simulink model "ModeInputHandle"  (R2018b)
settings: Solver=FixedStepDiscrete  StartTime=0.0  StopTime=10.0  FixedStep=0.01  RelTol=1e-3
undefined symbols (not defined in the file or in its folder): c, CmprtMdHMIReqExt2Tp1, CmprtMdHMIReqExtTp1, CmprtMdHMIReqTp1, d, e, EZESwReq1, f, g, IfVeSMSeStNumConfig, j, KeSMSuButtonLongPressedThrshldTm_Val, KeSMSuFoldType_Val, KeSMSwSeatSMSSeatMdTrigGapTimer_Val, KeSMSwSeatTrigWaitTimer_Val, KeSMSwSRSActiveValidTm_Val, LckUlckActvtFunc1, LstLckFunc1, LugSelectSw1, MdReqTp1, PowerMode1, SeatOccupiedSts1, SRSMode1, StPassCmprtMdCtrl_Md10_VCUConfig_Val, StPassCmprtMdCtrl_Md11_VCUConfig_Val, StPassCmprtMdCtrl_Md12_VCUConfig_Val, StPassCmprtMdCtrl_Md13_VCUConfig_Val, StPassCmprtMdCtrl_Md1_VCUConfig_Val, StPassCmprtMdCtrl_Md27_VCUConfig_Val, StPassCmprtMdCtrl_Md28_VCUConfig_Val, StPassCmprtMdCtrl_Md29_VCUConfig_Val, StPassCmprtMdCtrl_Md2_VCUConfig_Val, StPassCmprtMdCtrl_Md30_VCUConfig_Val, StPassCmprtMdCtrl_Md31_VCUConfig_Val, StPassCmprtMdCtrl_Md32_VCUConfig_Val, StPassCmprtMdCtrl_Md3_VCUConfig_Val, StPassCmprtMdCtrl_Md53_VCUConfig_Val, StPassCmprtMdCtrl_Md56_VCUConfig_Val, StPassCmprtMdCtrl_Md57_VCUConfig_Val, StPassCmprtMdCtrl_Md58_VCUConfig_Val, StPassCmprtMdCtrl_Md61_VCUConfig_Val, StPassCmprtMdCtrl_Md62_VCUConfig_Val, StPassCmprtMdCtrl_Md8_VCUConfig_Val, StPassCmprtMdCtrl_Md9_VCUConfig_Val, StSrv_StMd10_Config_Val, StSrv_StMd11_Config_Val, StSrv_StMd12_Config_Val, StSrv_StMd13_Config_Val, StSrv_StMd1_Config_Val, StSrv_StMd27_Config_Val, StSrv_StMd28_Config_Val, StSrv_StMd29_Config_Val, StSrv_StMd2_Config_Val, StSrv_StMd30_Config_Val, StSrv_StMd31_Config_Val, StSrv_StMd32_Config_Val, StSrv_StMd3_Config_Val, StSrv_StMd8_Config_Val, StSrv_StMd9_Config_Val, VehMovState1
libraries: MSMLib x91
(part 1 of 9)
settings Model: PauseTimes=0.13  Creator=su3dcu  LastModifiedBy=su3dcu
settings DataIOCC: SaveFormat=StructureWithTime  ReturnWorkspaceOutputs=on
settings OptimizationCC: DefaultParameterBehavior=Inlined  EnhancedBackFolding=on  PassReuseOutputArgsAs=Individual arguments  ZeroExternalMemoryAtStartup=off  ZeroInternalMemoryAtStartup=off  OptimizeBlockOrder=speed  DifferentSizesBufferReuse=on  OptimizationCustomize=off
settings DebuggingCC: ParameterTunabilityLossMsg=error
settings HardwareCC: ProdLongLongMode=on
settings ModelReferenceCC: ModelReferenceNumInstancesAllowed=Single
settings SFSimCC: SimCustomHeaderCode="#include\"Rte_Type.h\""  MATLABDynamicMemAlloc=off
settings RTWCC: SystemTargetFile=autosar.tlc  GenCodeOnly=on  TemplateMakefile=ert_default_tmf  Description=AUTOSAR  GenerateReport=on  BuildConfiguration=Debug  IncludeHyperlinkInReport=on  LaunchReport=on  CodeExecutionProfiling=on  GenerateTraceInfo=on  GenerateTraceReport=on  GenerateTraceReportSl=on  GenerateTraceReportSf=on  GenerateTraceReportEml=on  GenerateCodeMetricsReport=on
settings CodeAppCC: ForceParamTrailComments=on  IgnoreCustomStorageClasses=off  MaxIdLength=63  OperatorAnnotations=on  SimulinkDataObjDesc=on  SFDataObjDesc=on  InsertBlockDesc=on
settings STFCustomTargetCC: TargetLangStandard=C99 (ISO)  MultiwordLength=256  ParMdlRefBuildCompliant=on  CompOptLevelCompliant=on  IncludeMdlTerminateFcn=off  CombineOutputUpdateFcns=on  SuppressErrorStatus=on  ERTCustomFileBanners=on  SupportAbsoluteTime=off  PurelyIntegerCode=on  SupportNonFinite=off  SupportComplex=off  SupportContinuousTime=off  SupportNonInlinedSFcns=off  RemoveResetFunc=on  MATLABClassNameForMDSCustomization=Simulink.SoftwareTarget.ERTCustomization  AutosarCompliant=on  UseToolchainInfoCompliant=on  LookupTableObjectStructAxisOrder=2,1,3,4,...  LUTObjectStructOrderEvenSpacing=Size,Table,Breakpoints  SystemTargetFile=autosar.tlc
settings ERTTargetCC: TargetLangStandard=C99 (ISO)  ConcurrentExecutionCompliant=off  IncludeMdlTerminateFcn=off  SuppressErrorStatus=on  SupportAbsoluteTime=off  PurelyIntegerCode=on  SupportNonFinite=off  SupportComplex=off  ModelStepFunctionPrototypeControlCompliant=off  CPPClassGenCompliant=off  AutosarCompliant=on  LookupTableObjectStructAxisOrder=2,1,3,4,...  LUTObjectStructOrderEvenSpacing=Size,Table,Breakpoints  InlinedParameterPlacement=NonHierarchical  ERTCustomFileTemplate=example_file_process.tlc  ERTFilePackagingFormat=Compact
settings ConfigComp: DVTestSuiteOptimization=CombinedObjectives (Nonlinear Extended)  DVDetectActiveLogic=on  DVDetectOutOfBounds=on

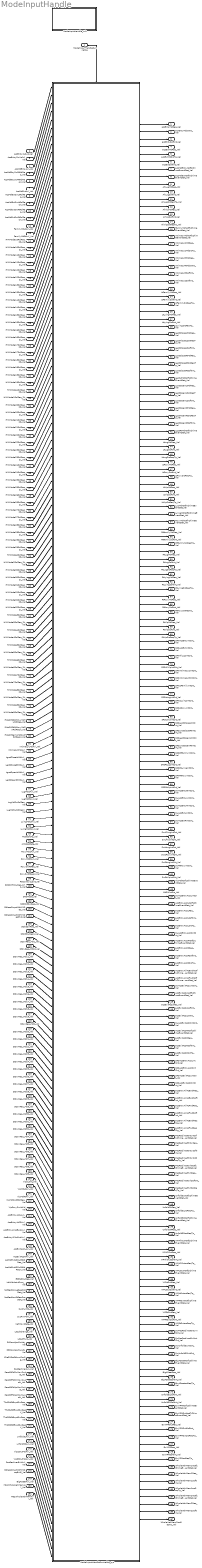
== system ModeInputHandle ==
  ModelInputHandleRunnable : Inport  SampleTime=0.01  OutputFunctionCall=on
  AcsEntry2LSwt_Val : Inport  Port=2  OutDataTypeStr=uint8  PortDimensions=1
  AcsEntrySwValid_Val : Inport  Port=3  OutDataTypeStr=uint8  PortDimensions=1
  AcsMdEntyAvl_Val : Inport  Port=4  OutDataTypeStr=boolean  PortDimensions=1
  AcsMdEtrySwRtRclReq_Val : Inport  Port=5  OutDataTypeStr=boolean  PortDimensions=1
  AcsMdEtrySwRtRclReqV_Val : Inport  Port=6  OutDataTypeStr=boolean  PortDimensions=1
  AcsMdExtAvl_Val : Inport  Port=7  OutDataTypeStr=boolean  PortDimensions=1
  AcsMdExtSwLtRclReq_Val : Inport  Port=8  OutDataTypeStr=boolean  PortDimensions=1
  AcsMdExtSwLtRclReqV_Val : Inport  Port=9  OutDataTypeStr=uint8  PortDimensions=1
  AcsMdExtSwRtRclReq_Val : Inport  Port=10  OutDataTypeStr=boolean  PortDimensions=1
  AcsMdExtSwRtRclReqV_Val : Inport  Port=11  OutDataTypeStr=boolean  PortDimensions=1
  FamilyMdLtAvl_Val : Inport  Port=12  OutDataTypeStr=boolean  PortDimensions=1
  FamilyMdRtAvl_Val : Inport  Port=13  OutDataTypeStr=boolean  PortDimensions=1
  HMIMode10RclReq_2R_Val : Inport  Port=14  OutDataTypeStr=Enum: MdReqTp1  PortDimensions=1
  HMIMode10RclReq_2L_Val : Inport  Port=15  OutDataTypeStr=Enum: MdReqTp1  PortDimensions=1
  HMIMode11RclReq_2R_Val : Inport  Port=16  OutDataTypeStr=Enum: MdReqTp1  PortDimensions=1
  HMIMode11RclReq_2L_Val : Inport  Port=17  OutDataTypeStr=Enum: MdReqTp1  PortDimensions=1
  HMIMode12RclReq_2R_Val : Inport  Port=18  OutDataTypeStr=Enum: MdReqTp1  PortDimensions=1
  HMIMode12RclReq_2L_Val : Inport  Port=19  OutDataTypeStr=Enum: MdReqTp1  PortDimensions=1
  HMIMode13RclReq_2R_Val : Inport  Port=20  OutDataTypeStr=Enum: MdReqTp1  PortDimensions=1
  HMIMode13RclReq_2L_Val : Inport  Port=21  OutDataTypeStr=Enum: MdReqTp1  PortDimensions=1
  HMIMode14RclReq_2R_Val : Inport  Port=22  OutDataTypeStr=Enum: MdReqTp1  PortDimensions=1
  HMIMode14RclReq_2L_Val : Inport  Port=23  OutDataTypeStr=Enum: MdReqTp1  PortDimensions=1
  HMIMode15RclReq_2R_Val : Inport  Port=24  OutDataTypeStr=Enum: MdReqTp1  PortDimensions=1
  HMIMode15RclReq_2L_Val : Inport  Port=25  OutDataTypeStr=Enum: MdReqTp1  PortDimensions=1
  HMIMode16RclReq_2R_Val : Inport  Port=26  OutDataTypeStr=Enum: MdReqTp1  PortDimensions=1
  HMIMode16RclReq_2L_Val : Inport  Port=27  OutDataTypeStr=Enum: MdReqTp1  PortDimensions=1
  HMIMode17RclReq_2R_Val : Inport  Port=28  OutDataTypeStr=Enum: MdReqTp1  PortDimensions=1
  HMIMode17RclReq_2L_Val : Inport  Port=29  OutDataTypeStr=Enum: MdReqTp1  PortDimensions=1
  HMIMode18RclReq_2R_Val : Inport  Port=30  OutDataTypeStr=Enum: MdReqTp1  PortDimensions=1
  HMIMode18RclReq_2L_Val : Inport  Port=31  OutDataTypeStr=Enum: MdReqTp1  PortDimensions=1
  HMIMode19RclReq_2R_Val : Inport  Port=32  OutDataTypeStr=Enum: MdReqTp1  PortDimensions=1
  HMIMode19RclReq_2L_Val : Inport  Port=33  OutDataTypeStr=Enum: MdReqTp1  PortDimensions=1
  HMIMode1RclReq_2R_Val : Inport  Port=34  OutDataTypeStr=Enum: MdReqTp1  PortDimensions=1
  HMIMode1RclReq_2L_Val : Inport  Port=35  OutDataTypeStr=Enum: MdReqTp1  PortDimensions=1
  HMIMode20RclReq_2R_Val : Inport  Port=36  OutDataTypeStr=Enum: MdReqTp1  PortDimensions=1
  HMIMode20RclReq_2L_Val : Inport  Port=37  OutDataTypeStr=Enum: MdReqTp1  PortDimensions=1
  HMIMode21RclReq_2R_Val : Inport  Port=38  OutDataTypeStr=Enum: MdReqTp1  PortDimensions=1
  HMIMode21RclReq_2L_Val : Inport  Port=39  OutDataTypeStr=Enum: MdReqTp1  PortDimensions=1
  HMIMode22RclReq_2R_Val : Inport  Port=40  OutDataTypeStr=Enum: MdReqTp1  PortDimensions=1
  HMIMode22RclReq_2L_Val : Inport  Port=41  OutDataTypeStr=Enum: MdReqTp1  PortDimensions=1
  HMIMode23RclReq_2R_Val : Inport  Port=42  OutDataTypeStr=Enum: MdReqTp1  PortDimensions=1
  HMIMode23RclReq_2L_Val : Inport  Port=43  OutDataTypeStr=Enum: MdReqTp1  PortDimensions=1
  HMIMode24RclReq_2R_Val : Inport  Port=44  OutDataTypeStr=Enum: MdReqTp1  PortDimensions=1
  HMIMode24RclReq_2L_Val : Inport  Port=45  OutDataTypeStr=Enum: MdReqTp1  PortDimensions=1
  HMIMode25RclReq_2R_Val : Inport  Port=46  OutDataTypeStr=Enum: MdReqTp1  PortDimensions=1
  HMIMode25RclReq_2L_Val : Inport  Port=47  OutDataTypeStr=Enum: MdReqTp1  PortDimensions=1
  HMIMode26RclReq_2R_Val : Inport  Port=48  OutDataTypeStr=Enum: MdReqTp1  PortDimensions=1
  HMIMode26RclReq_2L_Val : Inport  Port=49  OutDataTypeStr=Enum: MdReqTp1  PortDimensions=1
  HMIMode27RclReq_2R_Val : Inport  Port=50  OutDataTypeStr=Enum: MdReqTp1  PortDimensions=1
  HMIMode27RclReq_2L_Val : Inport  Port=51  OutDataTypeStr=Enum: MdReqTp1  PortDimensions=1
  HMIMode28RclReq_2R_Val : Inport  Port=52  OutDataTypeStr=Enum: MdReqTp1  PortDimensions=1
  HMIMode28RclReq_2L_Val : Inport  Port=53  OutDataTypeStr=Enum: MdReqTp1  PortDimensions=1
  HMIMode29RclReq_2R_Val : Inport  Port=54  OutDataTypeStr=Enum: MdReqTp1  PortDimensions=1
  HMIMode29RclReq_2L_Val : Inport  Port=55  OutDataTypeStr=Enum: MdReqTp1  PortDimensions=1
  HMIMode2RclReq_2R_Val : Inport  Port=56  OutDataTypeStr=Enum: MdReqTp1  PortDimensions=1
  HMIMode2RclReq_2L_Val : Inport  Port=57  OutDataTypeStr=Enum: MdReqTp1  PortDimensions=1
  HMIMode30RclReq_2R_Val : Inport  Port=58  OutDataTypeStr=Enum: MdReqTp1  PortDimensions=1
  HMIMode30RclReq_2L_Val : Inport  Port=59  OutDataTypeStr=Enum: MdReqTp1  PortDimensions=1
  HMIMode31RclReq_2R_Val : Inport  Port=60  OutDataTypeStr=Enum: MdReqTp1  PortDimensions=1
  HMIMode31RclReq_2L_Val : Inport  Port=61  OutDataTypeStr=Enum: MdReqTp1  PortDimensions=1
  HMIMode32RclReq_2R_Val : Inport  Port=62  OutDataTypeStr=Enum: MdReqTp1  PortDimensions=1
  HMIMode32RclReq_2L_Val : Inport  Port=63  OutDataTypeStr=Enum: MdReqTp1  PortDimensions=1
  HMIMode3RclReq_2R_Val : Inport  Port=64  OutDataTypeStr=Enum: MdReqTp1  PortDimensions=1
  HMIMode3RclReq_2L_Val : Inport  Port=65  OutDataTypeStr=Enum: MdReqTp1  PortDimensions=1
  HMIMode4RclReq_2R_Val : Inport  Port=66  OutDataTypeStr=Enum: MdReqTp1  PortDimensions=1
  HMIMode4RclReq_2L_Val : Inport  Port=67  OutDataTypeStr=Enum: MdReqTp1  PortDimensions=1
  HMIMode5RclReq_2R_Val : Inport  Port=68  OutDataTypeStr=Enum: MdReqTp1  PortDimensions=1
  HMIMode5RclReq_2L_Val : Inport  Port=69  OutDataTypeStr=Enum: MdReqTp1  PortDimensions=1
  HMIMode6RclReq_2R_Val : Inport  Port=70  OutDataTypeStr=Enum: MdReqTp1  PortDimensions=1
  HMIMode6RclReq_2L_Val : Inport  Port=71  OutDataTypeStr=Enum: MdReqTp1  PortDimensions=1
  HMIMode7RclReq_2R_Val : Inport  Port=72  OutDataTypeStr=Enum: MdReqTp1  PortDimensions=1
  HMIMode7RclReq_2L_Val : Inport  Port=73  OutDataTypeStr=Enum: MdReqTp1  PortDimensions=1
  HMIMode8RclReq_2R_Val : Inport  Port=74  OutDataTypeStr=Enum: MdReqTp1  PortDimensions=1
  HMIMode8RclReq_2L_Val : Inport  Port=75  OutDataTypeStr=Enum: MdReqTp1  PortDimensions=1
  HMIMode9RclReq_2R_Val : Inport  Port=76  OutDataTypeStr=Enum: MdReqTp1  PortDimensions=1
  HMIMode9RclReq_2L_Val : Inport  Port=77  OutDataTypeStr=Enum: MdReqTp1  PortDimensions=1
  IfVeSMSbRrRcvyMdSwRclReq_Val : Inport  Port=78  OutDataTypeStr=uint8  PortDimensions=1
  IfVeSMSbRrRcvyMdSwRclReqV_Val : Inport  Port=79  OutDataTypeStr=boolean  PortDimensions=1
  IfVeSMSeVipMdSwRtRclReqV_Val : Inport  Port=80  OutDataTypeStr=boolean  PortDimensions=1
  IntimacyLMdAvl_Val : Inport  Port=81  OutDataTypeStr=boolean  PortDimensions=1
  IntimacyRMdAvl_Val : Inport  Port=82  OutDataTypeStr=boolean  PortDimensions=1
  LgrstCloseLtMdAvl_Val : Inport  Port=83  OutDataTypeStr=boolean  PortDimensions=1
  LgrstCloseRtMdAvl_Val : Inport  Port=84  OutDataTypeStr=boolean  PortDimensions=1
  LgrstOpenLtMdAvl_Val : Inport  Port=85  OutDataTypeStr=boolean  PortDimensions=1
  LgrstOpenRtMdAvl_Val : Inport  Port=86  OutDataTypeStr=boolean  PortDimensions=1
  LugMdLtAvl_Val : Inport  Port=87  OutDataTypeStr=boolean  PortDimensions=1
  LugMdRtAvl_Val : Inport  Port=88  OutDataTypeStr=boolean  PortDimensions=1
  LugMdSwRclReq_Val : Inport  Port=89  OutDataTypeStr=boolean  PortDimensions=1
  LugMdSwRclReqV_Val : Inport  Port=90  OutDataTypeStr=uint8  PortDimensions=1
  LyingMdLtAvl_Val : Inport  Port=91  OutDataTypeStr=boolean  PortDimensions=1
  LyingMdRtAvl_Val : Inport  Port=92  OutDataTypeStr=boolean  PortDimensions=1
  ModeSrcTp_Val : Inport  Port=93  OutDataTypeStr=Enum: SrcReqTp1  PortDimensions=1
  oModeState_Val : Inport  Port=94  OutDataTypeStr=Enum: MdTp1  PortDimensions=1
  RcvyMdLtAvl_Val : Inport  Port=95  OutDataTypeStr=boolean  PortDimensions=1
  RcvyMdRtAvl_Val : Inport  Port=96  OutDataTypeStr=boolean  PortDimensions=1
  RcvySwRtReq_Val : Inport  Port=97  OutDataTypeStr=boolean  PortDimensions=1
  RcvySwRtReqV_Val : Inport  Port=98  OutDataTypeStr=boolean  PortDimensions=1
  Recovery2LSwt_Val : Inport  Port=99  OutDataTypeStr=uint8  PortDimensions=1
  SRSCnfmSwReq_67_2_Val : Inport  Port=100  OutDataTypeStr=boolean  PortDimensions=1
  SRSMode_Val : Inport  Port=101  OutDataTypeStr=Enum: SRSCurMode1  PortDimensions=1
  SRSSlctSwReq_Val : Inport  Port=102  OutDataTypeStr=Enum: SRSMode1  PortDimensions=1
  StPassCmprtMdHMIReq_Val : Inport  Port=103  OutDataTypeStr=Enum: CmprtMdHMIReqTp1  PortDimensions=1
  StPassCmprtMdHMIReqExt_Val : Inport  Port=104  OutDataTypeStr=Enum: CmprtMdHMIReqExtTp1  PortDimensions=1
  StSlctSwReq_Val : Inport  Port=105  OutDataTypeStr=Enum: LugSelectSw1  PortDimensions=1
  StSlctSwReqV_Val : Inport  Port=106  OutDataTypeStr=boolean  PortDimensions=1
  StSrvReq_Md1_Val : Inport  Port=107  OutDataTypeStr=boolean  PortDimensions=1
  StSrvReq_Md10_Val : Inport  Port=108  OutDataTypeStr=boolean  PortDimensions=1
  StSrvReq_Md11_Val : Inport  Port=109  OutDataTypeStr=boolean  PortDimensions=1
  StSrvReq_Md12_Val : Inport  Port=110  OutDataTypeStr=boolean  PortDimensions=1
  StSrvReq_Md13_Val : Inport  Port=111  OutDataTypeStr=boolean  PortDimensions=1
  StSrvReq_Md14_Val : Inport  Port=112  OutDataTypeStr=boolean  PortDimensions=1
  StSrvReq_Md15_Val : Inport  Port=113  OutDataTypeStr=boolean  PortDimensions=1
  StSrvReq_Md16_Val : Inport  Port=114  OutDataTypeStr=boolean  PortDimensions=1
  StSrvReq_Md17_Val : Inport  Port=115  OutDataTypeStr=boolean  PortDimensions=1
  StSrvReq_Md18_Val : Inport  Port=116  OutDataTypeStr=boolean  PortDimensions=1
  StSrvReq_Md19_Val : Inport  Port=117  OutDataTypeStr=boolean  PortDimensions=1
  StSrvReq_Md2_Val : Inport  Port=118  OutDataTypeStr=boolean  PortDimensions=1
  StSrvReq_Md20_Val : Inport  Port=119  OutDataTypeStr=boolean  PortDimensions=1
  StSrvReq_Md21_Val : Inport  Port=120  OutDataTypeStr=boolean  PortDimensions=1
  StSrvReq_Md22_Val : Inport  Port=121  OutDataTypeStr=boolean  PortDimensions=1
  StSrvReq_Md23_Val : Inport  Port=122  OutDataTypeStr=boolean  PortDimensions=1
  StSrvReq_Md24_Val : Inport  Port=123  OutDataTypeStr=boolean  PortDimensions=1
  StSrvReq_Md25_Val : Inport  Port=124  OutDataTypeStr=boolean  PortDimensions=1
  StSrvReq_Md26_Val : Inport  Port=125  OutDataTypeStr=boolean  PortDimensions=1
  StSrvReq_Md27_Val : Inport  Port=126  OutDataTypeStr=boolean  PortDimensions=1
  StSrvReq_Md28_Val : Inport  Port=127  OutDataTypeStr=boolean  PortDimensions=1
  StSrvReq_Md29_Val : Inport  Port=128  OutDataTypeStr=boolean  PortDimensions=1
  StSrvReq_Md3_Val : Inport  Port=129  OutDataTypeStr=boolean  PortDimensions=1
  StSrvReq_Md30_Val : Inport  Port=130  OutDataTypeStr=boolean  PortDimensions=1
  StSrvReq_Md31_Val : Inport  Port=131  OutDataTypeStr=boolean  PortDimensions=1
  StSrvReq_Md32_Val : Inport  Port=132  OutDataTypeStr=boolean  PortDimensions=1
  StSrvReq_Md4_Val : Inport  Port=133  OutDataTypeStr=boolean  PortDimensions=1
  StSrvReq_Md5_Val : Inport  Port=134  OutDataTypeStr=boolean  PortDimensions=1
  StSrvReq_Md6_Val : Inport  Port=135  OutDataTypeStr=boolean  PortDimensions=1
  StSrvReq_Md7_Val : Inport  Port=136  OutDataTypeStr=boolean  PortDimensions=1
  StSrvReq_Md8_Val : Inport  Port=137  OutDataTypeStr=boolean  PortDimensions=1
  StSrvReq_Md9_Val : Inport  Port=138  OutDataTypeStr=boolean  PortDimensions=1
  Vip2LSwt_Val : Inport  Port=139  OutDataTypeStr=uint8  PortDimensions=1
  VipMdLtAvl_Val : Inport  Port=140  OutDataTypeStr=boolean  PortDimensions=1
  VipMdRtAvl_Val : Inport  Port=141  OutDataTypeStr=boolean  PortDimensions=1
  VipMdSwRtRclReq_Val : Inport  Port=142  OutDataTypeStr=boolean  PortDimensions=1
  VipRcvySwValid_Val : Inport  Port=143  OutDataTypeStr=uint8  PortDimensions=1
  AcsEntry4s2LAvl_Val : Inport  Port=144  OutDataTypeStr=boolean  PortDimensions=1
  AcsEntry4s2RAvl_Val : Inport  Port=145  OutDataTypeStr=boolean  PortDimensions=1
  AcsEntryAll4sBwdAvl_Val : Inport  Port=146  OutDataTypeStr=boolean  PortDimensions=1
  AcsEntryAll4sFwdAvl_Val : Inport  Port=147  OutDataTypeStr=boolean  PortDimensions=1
  AcsExit4s2LAvl_Val : Inport  Port=148  OutDataTypeStr=boolean  PortDimensions=1
  AcsExit4s2RAvl_Val : Inport  Port=149  OutDataTypeStr=boolean  PortDimensions=1
  AcsMdExt4SSwRtRclReq_Val : Inport  Port=150  OutDataTypeStr=boolean  PortDimensions=1
  AcsMdExt4SSwRtRclReqV_Val : Inport  Port=151  OutDataTypeStr=boolean  PortDimensions=1
  EZE4SSwReq_Val : Inport  Port=152  OutDataTypeStr=Enum: EZESwReq1  PortDimensions=1
  LckUlckActvtFunc_Val : Inport  Port=153  OutDataTypeStr=Enum: LckUlckActvtFunc1  PortDimensions=1
  NotSecRowLeSeaOccStat_Val : Inport  Port=154  OutDataTypeStr=Enum: SeatOccupiedSts1  PortDimensions=1
  NotSecRowRtSeaOccStat_Val : Inport  Port=155  OutDataTypeStr=Enum: SeatOccupiedSts1  PortDimensions=1
  SysPwrMd_Val : Inport  Port=156  OutDataTypeStr=Enum: PowerMode1  PortDimensions=1
  SysPwrMdV_Val : Inport  Port=157  OutDataTypeStr=boolean  PortDimensions=1
  VehMovState_Val : Inport  Port=158  OutDataTypeStr=Enum: VehMovState1  PortDimensions=1
  LstLckChange_Val : Inport  Port=159  OutDataTypeStr=uint8  PortDimensions=1
  LstLckFunc_Val : Inport  Port=160  OutDataTypeStr=Enum: LstLckFunc1  PortDimensions=1
  RLDoorAjarSwAct_Val : Inport  Port=161  OutDataTypeStr=boolean  PortDimensions=1
  RRDoorAjarSwAct_Val : Inport  Port=162  OutDataTypeStr=boolean  PortDimensions=1
  IfVeSMSeStNumConfig_Val : Inport  Port=163  OutDataTypeStr=Enum: IfVeSMSeStNumConfig  PortDimensions=1
  PasReclinerAvl_Val : Inport  Port=164  OutDataTypeStr=boolean  PortDimensions=1
  PassStFldDnMovSwAct_Val : Inport  Port=165  OutDataTypeStr=boolean  PortDimensions=1
  PassStFldDnMovSwActV_Val : Inport  Port=166  OutDataTypeStr=boolean  PortDimensions=1
  PassStFldUpMovSwAct_Val : Inport  Port=167  OutDataTypeStr=boolean  PortDimensions=1
  PassStFldUpMovSwActV_Val : Inport  Port=168  OutDataTypeStr=boolean  PortDimensions=1
  ThdRLtStExpdSwReq_Val : Inport  Port=169  OutDataTypeStr=boolean  PortDimensions=1
  ThdRLtStExpdSwReqV_Val : Inport  Port=170  OutDataTypeStr=boolean  PortDimensions=1
  ThdRRtStExpdSwReq_Val : Inport  Port=171  OutDataTypeStr=boolean  PortDimensions=1
  ThdRRtStExpdSwReqV_Val : Inport  Port=172  OutDataTypeStr=boolean  PortDimensions=1
  unfold3LAvl_Val : Inport  Port=173  OutDataTypeStr=boolean  PortDimensions=1
  unfold3RAvl_Val : Inport  Port=174  OutDataTypeStr=boolean  PortDimensions=1
  VipLtOutMdAvl_Val : Inport  Port=175  OutDataTypeStr=boolean  PortDimensions=1
  VipRtOutMdAvl_Val : Inport  Port=176  OutDataTypeStr=boolean  PortDimensions=1
  PasReclinerExitAvl_Val : Inport  Port=177  OutDataTypeStr=boolean  PortDimensions=1
  StPassCmprtMdHMIReqExt2_Val : Inport  Port=178  OutDataTypeStr=Enum: CmprtMdHMIReqExt2Tp1  PortDimensions=1
  Big4SeatAvl_Val : Inport  Port=179  OutDataTypeStr=boolean  PortDimensions=1
  M61WholeVehMemAvl_Val : Inport  Port=180  OutDataTypeStr=boolean  PortDimensions=1
  M62WholeVehMemAvl_Val : Inport  Port=181  OutDataTypeStr=boolean  PortDimensions=1
  ModeInputHandle_Init : Subsystem
  ModelInputHandleRunnable_sys : Subsystem
  acsEntyMdReq_Val : Outport  OutDataTypeStr=boolean  PortDimensions=1
  acsEntyMdSrcTp_Val : Outport  Port=2  OutDataTypeStr=Enum: SrcReqTp1  PortDimensions=1
  acsEntySoftInt_Val : Outport  Port=3  OutDataTypeStr=IntEnable  PortDimensions=1
  acsExtMdReq_Val : Outport  Port=4  OutDataTypeStr=boolean  PortDimensions=1
  acsExtMdSrcTp_Val : Outport  Port=5  OutDataTypeStr=Enum: SrcReqTp1  PortDimensions=1
  acsExtSoftInt_Val : Outport  Port=6  OutDataTypeStr=IntEnable  PortDimensions=1
  acsMdEntryNotf1ChimeEventStat_Val : Outport  Port=7  OutDataTypeStr=boolean  PortDimensions=1
  acsMdExtNotf1ChimeEventStat_Val : Outport  Port=8  OutDataTypeStr=boolean  PortDimensions=1
  AllLugMdReq_Val : Outport  Port=9  OutDataTypeStr=boolean  PortDimensions=1
  AllLugSoftInt_Val : Outport  Port=10  OutDataTypeStr=IntEnable  PortDimensions=1
  AllLugSrcReqTp_Val : Outport  Port=11  OutDataTypeStr=Enum: SrcReqTp1  PortDimensions=1
  AllVipMdReq_Val : Outport  Port=12  OutDataTypeStr=boolean  PortDimensions=1
  AllVipSoftInt_Val : Outport  Port=13  OutDataTypeStr=IntEnable  PortDimensions=1
  AllVipSrcReqTp_Val : Outport  Port=14  OutDataTypeStr=Enum: SrcReqTp1  PortDimensions=1
  FamilyMdNotf1ChimeEventStat_Val : Outport  Port=15  OutDataTypeStr=boolean  PortDimensions=1
  IntimacyMdNotf1ChimeEventStat_Val : Outport  Port=16  OutDataTypeStr=boolean  PortDimensions=1
  IntimacyLtMdReq_Val : Outport  Port=17  OutDataTypeStr=boolean  PortDimensions=1
  IntimacyLtMdSrcTp_Val : Outport  Port=18  OutDataTypeStr=Enum: SrcReqTp1  PortDimensions=1
  IntimacyRtMdReq_Val : Outport  Port=19  OutDataTypeStr=boolean  PortDimensions=1
  IntimacyRtMdSrcTp_Val : Outport  Port=20  OutDataTypeStr=Enum: SrcReqTp1  PortDimensions=1
  IntimacyRtSoftInt_Val : Outport  Port=21  OutDataTypeStr=IntEnable  PortDimensions=1
  IntimacyLtSoftInt_Val : Outport  Port=22  OutDataTypeStr=IntEnable  PortDimensions=1
  LtFamilyMdReq_Val : Outport  Port=23  OutDataTypeStr=boolean  PortDimensions=1
  LtFamilySoftInt_Val : Outport  Port=24  OutDataTypeStr=IntEnable  PortDimensions=1
  LtFamilySrcReqTp_Val : Outport  Port=25  OutDataTypeStr=Enum: SrcReqTp1  PortDimensions=1
  LtLyingMdReq_Val : Outport  Port=26  OutDataTypeStr=boolean  PortDimensions=1
  LtLyingSoftInt_Val : Outport  Port=27  OutDataTypeStr=IntEnable  PortDimensions=1
  LtLyingSrcReqTp_Val : Outport  Port=28  OutDataTypeStr=Enum: SrcReqTp1  PortDimensions=1
  LgrstCloseLtMdReq_Val : Outport  Port=29  OutDataTypeStr=boolean  PortDimensions=1
  LgrstCloseLtSrcReqTp_Val : Outport  Port=30  OutDataTypeStr=Enum: SrcReqTp1  PortDimensions=1
  LgrstCloseLtSoftInt_Val : Outport  Port=31  OutDataTypeStr=IntEnable  PortDimensions=1
  LgrstCloseRtMdReq_Val : Outport  Port=32  OutDataTypeStr=boolean  PortDimensions=1
  LgrstCloseRtSrcReqTp_Val : Outport  Port=33  OutDataTypeStr=Enum: SrcReqTp1  PortDimensions=1
  LgrstCloseRtSoftInt_Val : Outport  Port=34  OutDataTypeStr=IntEnable  PortDimensions=1
  LgrstLtMdNotf1ChimeEventStat_Val : Outport  Port=35  OutDataTypeStr=boolean  PortDimensions=1
  LgrstOpenLtMdReq_Val : Outport  Port=36  OutDataTypeStr=boolean  PortDimensions=1
  LgrstOpenLtSrcReqTp_Val : Outport  Port=37  OutDataTypeStr=Enum: SrcReqTp1  PortDimensions=1
  LgrstOpenLtSoftInt_Val : Outport  Port=38  OutDataTypeStr=IntEnable  PortDimensions=1
  LgrstOpenRtMdReq_Val : Outport  Port=39  OutDataTypeStr=boolean  PortDimensions=1
  LgrstOpenRtSrcReqTp_Val : Outport  Port=40  OutDataTypeStr=Enum: SrcReqTp1  PortDimensions=1
  LgrstOpenRtSoftInt_Val : Outport  Port=41  OutDataTypeStr=IntEnable  PortDimensions=1
  LgrstRtMdNotf1ChimeEventStat_Val : Outport  Port=42  OutDataTypeStr=boolean  PortDimensions=1
  LtLugMdReq_Val : Outport  Port=43  OutDataTypeStr=boolean  PortDimensions=1
  LtLugSoftInt_Val : Outport  Port=44  OutDataTypeStr=IntEnable  PortDimensions=1
  LtLugSrcReqTp_Val : Outport  Port=45  OutDataTypeStr=Enum: SrcReqTp1  PortDimensions=1
  LtRcvyMdReq_Val : Outport  Port=46  OutDataTypeStr=boolean  PortDimensions=1
  LtRcvySoftInt_Val : Outport  Port=47  OutDataTypeStr=IntEnable  PortDimensions=1
  LtRcvySrcReqTp_Val : Outport  Port=48  OutDataTypeStr=Enum: SrcReqTp1  PortDimensions=1
  LtVipMdReq_Val : Outport  Port=49  OutDataTypeStr=boolean  PortDimensions=1
  LtVipSoftInt_Val : Outport  Port=50  OutDataTypeStr=IntEnable  PortDimensions=1
  LtVipSrcReqTp_Val : Outport  Port=51  OutDataTypeStr=Enum: SrcReqTp1  PortDimensions=1
  LugMdNotf1ChimeEventStat_Val : Outport  Port=52  OutDataTypeStr=boolean  PortDimensions=1
  LyingMdNotf1ChimeEventStat_Val : Outport  Port=53  OutDataTypeStr=boolean  PortDimensions=1
  RcvyMdNotf1ChimeEventStat_Val : Outport  Port=54  OutDataTypeStr=boolean  PortDimensions=1
  RtFamilyMdReq_Val : Outport  Port=55  OutDataTypeStr=boolean  PortDimensions=1
  RtFamilySoftInt_Val : Outport  Port=56  OutDataTypeStr=IntEnable  PortDimensions=1
  RtFamilySrcReqTp_Val : Outport  Port=57  OutDataTypeStr=Enum: SrcReqTp1  PortDimensions=1
  RtLugMdReq_Val : Outport  Port=58  OutDataTypeStr=boolean  PortDimensions=1
  RtLugSoftInt_Val : Outport  Port=59  OutDataTypeStr=IntEnable  PortDimensions=1
  RtLugSrcReqTp_Val : Outport  Port=60  OutDataTypeStr=Enum: SrcReqTp1  PortDimensions=1
  RtLyingMdReq_Val : Outport  Port=61  OutDataTypeStr=boolean  PortDimensions=1
  RtLyingSoftInt_Val : Outport  Port=62  OutDataTypeStr=IntEnable  PortDimensions=1
  RtLyingSrcReqTp_Val : Outport  Port=63  OutDataTypeStr=Enum: SrcReqTp1  PortDimensions=1
  RtRcvyMdReq_Val : Outport  Port=64  OutDataTypeStr=boolean  PortDimensions=1
  RtRcvySoftInt_Val : Outport  Port=65  OutDataTypeStr=IntEnable  PortDimensions=1
  RtRcvySrcReqTp_Val : Outport  Port=66  OutDataTypeStr=Enum: SrcReqTp1  PortDimensions=1
  RtVipMdReq_Val : Outport  Port=67  OutDataTypeStr=boolean  PortDimensions=1
  RtVipSoftInt_Val : Outport  Port=68  OutDataTypeStr=IntEnable  PortDimensions=1
  RtVipSrcReqTp_Val : Outport  Port=69  OutDataTypeStr=Enum: SrcReqTp1  PortDimensions=1
  SRSAcsEntyIntCnt_Val : Outport  Port=70  OutDataTypeStr=IntCnt  PortDimensions=1
  SRSAcsExtIntCnt_Val : Outport  Port=71  OutDataTypeStr=IntCnt  PortDimensions=1
  SRSAllLugIntCnt_Val : Outport  Port=72  OutDataTypeStr=IntCnt  PortDimensions=1
  SRSAllVipIntCnt_Val : Outport  Port=73  OutDataTypeStr=IntCnt  PortDimensions=1
  SRSIntimacyLtIntCnt_Val : Outport  Port=74  OutDataTypeStr=IntCnt  PortDimensions=1
  SRSIntimacyRtIntCnt_Val : Outport  Port=75  OutDataTypeStr=IntCnt  PortDimensions=1
  SRSLtFamilyIntCnt_Val : Outport  Port=76  OutDataTypeStr=IntCnt  PortDimensions=1
  SRSLtLugIntCnt_Val : Outport  Port=77  OutDataTypeStr=IntCnt  PortDimensions=1
  SRSLtLyingIntCnt_Val : Outport  Port=78  OutDataTypeStr=IntCnt  PortDimensions=1
  SRSLtRcvyIntCnt_Val : Outport  Port=79  OutDataTypeStr=IntCnt  PortDimensions=1
  SRSLtVipIntCnt_Val : Outport  Port=80  OutDataTypeStr=IntCnt  PortDimensions=1
  SRSLgrstCloseLtIntCnt_Val : Outport  Port=81  OutDataTypeStr=IntCnt  PortDimensions=1
  SRSLgrstCloseRtIntCnt_Val : Outport  Port=82  OutDataTypeStr=IntCnt  PortDimensions=1
  SRSLgrstOpenLtIntCnt_Val : Outport  Port=83  OutDataTypeStr=IntCnt  PortDimensions=1
  SRSLgrstOpenRtIntCnt_Val : Outport  Port=84  OutDataTypeStr=IntCnt  PortDimensions=1
  SRSRtFamilyIntCnt_Val : Outport  Port=85  OutDataTypeStr=IntCnt  PortDimensions=1
  SRSRtLugIntCnt_Val : Outport  Port=86  OutDataTypeStr=IntCnt  PortDimensions=1
  SRSRtLyingIntCnt_Val : Outport  Port=87  OutDataTypeStr=IntCnt  PortDimensions=1
  SRSRtRcvyIntCnt_Val : Outport  Port=88  OutDataTypeStr=IntCnt  PortDimensions=1
  SRSRtVipIntCnt_Val : Outport  Port=89  OutDataTypeStr=IntCnt  PortDimensions=1
  SwAcsEntyBIntCnt_Val : Outport  Port=90  OutDataTypeStr=IntCnt  PortDimensions=1
  SwAcsEntyLIntCnt_Val : Outport  Port=91  OutDataTypeStr=IntCnt  PortDimensions=1
  SwAcsEntyRIntCnt_Val : Outport  Port=92  OutDataTypeStr=IntCnt  PortDimensions=1
  SwAcsExtLIntCnt_Val : Outport  Port=93  OutDataTypeStr=IntCnt  PortDimensions=1
  SwAcsExtRIntCnt_Val : Outport  Port=94  OutDataTypeStr=IntCnt  PortDimensions=1
  SwAllLugIntCnt_Val : Outport  Port=95  OutDataTypeStr=IntCnt  PortDimensions=1
  SwLfVipIntCnt_Val : Outport  Port=96  OutDataTypeStr=IntCnt  PortDimensions=1
  SwLtLugIntCnt_Val : Outport  Port=97  OutDataTypeStr=IntCnt  PortDimensions=1
  SwLtRcvyIntCnt_Val : Outport  Port=98  OutDataTypeStr=IntCnt  PortDimensions=1
  SwRtLugIntCnt_Val : Outport  Port=99  OutDataTypeStr=IntCnt  PortDimensions=1
  SwRtRcvyIntCnt_Val : Outport  Port=100  OutDataTypeStr=IntCnt  PortDimensions=1
  SwRtVipIntCnt_Val : Outport  Port=101  OutDataTypeStr=IntCnt  PortDimensions=1
  VipMdNotf1ChimeEventStat_Val : Outport  Port=102  OutDataTypeStr=boolean  PortDimensions=1
  MdSWIntSrc_Val : Outport  Port=103  OutDataTypeStr=uint16  PortDimensions=1
  SwAcsEntry4s2LIntCnt_Val : Outport  Port=104  OutDataTypeStr=IntCnt  PortDimensions=1
  AcsEntry4s2LNotf1ChimeEventStat_Val : Outport  Port=105  OutDataTypeStr=boolean  PortDimensions=1
  acsEntry4s2LReq_Val : Outport  Port=106  OutDataTypeStr=boolean  PortDimensions=1
  acsEntry4s2LSoftInt_Val : Outport  Port=107  OutDataTypeStr=IntEnable  PortDimensions=1
  acsEntry4s2LSrcTp_Val : Outport  Port=108  OutDataTypeStr=Enum: SrcReqTp1  PortDimensions=1
  SwAcsEntry4s2RIntCnt_Val : Outport  Port=109  OutDataTypeStr=IntCnt  PortDimensions=1
  AcsEntry4s2RNotf1ChimeEventStat_Val : Outport  Port=110  OutDataTypeStr=boolean  PortDimensions=1
  acsEntry4s2RReq_Val : Outport  Port=111  OutDataTypeStr=boolean  PortDimensions=1
  acsEntry4s2RSoftInt_Val : Outport  Port=112  OutDataTypeStr=IntEnable  PortDimensions=1
  acsEntry4s2RSrcTp_Val : Outport  Port=113  OutDataTypeStr=Enum: SrcReqTp1  PortDimensions=1
  AcsEntryAll4sBwdNotf1ChimeEventStat_Val : Outport  Port=114  OutDataTypeStr=boolean  PortDimensions=1
  AcsEntryAll4sFwdNotf1ChimeEventStat_Val : Outport  Port=115  OutDataTypeStr=boolean  PortDimensions=1
  SwAcsExit4s2LIntCnt_Val : Outport  Port=116  OutDataTypeStr=IntCnt  PortDimensions=1
  AcsExit4s2LNotf1ChimeEventStat_Val : Outport  Port=117  OutDataTypeStr=boolean  PortDimensions=1
  acsExit4s2LReq_Val : Outport  Port=118  OutDataTypeStr=boolean  PortDimensions=1
  acsExit4s2LSoftInt_Val : Outport  Port=119  OutDataTypeStr=IntEnable  PortDimensions=1
  acsExit4s2LSrcTp_Val : Outport  Port=120  OutDataTypeStr=Enum: SrcReqTp1  PortDimensions=1
  SwAcsExit4s2RIntCnt_Val : Outport  Port=121  OutDataTypeStr=IntCnt  PortDimensions=1
  AcsExit4s2RNotf1ChimeEventStat_Val : Outport  Port=122  OutDataTypeStr=boolean  PortDimensions=1
  acsExit4s2RReq_Val : Outport  Port=123  OutDataTypeStr=boolean  PortDimensions=1
  acsExit4s2RSoftInt_Val : Outport  Port=124  OutDataTypeStr=IntEnable  PortDimensions=1
  acsExit4s2RSrcTp_Val : Outport  Port=125  OutDataTypeStr=Enum: SrcReqTp1  PortDimensions=1
  SRSAcsEntry4s2LIntCnt_Val : Outport  Port=126  OutDataTypeStr=IntCnt  PortDimensions=1
  SRSAcsEntry4s2RIntCnt_Val : Outport  Port=127  OutDataTypeStr=IntCnt  PortDimensions=1
  SRSAcsExit4s2LIntCnt_Val : Outport  Port=128  OutDataTypeStr=IntCnt  PortDimensions=1
  SRSAcsExit4s2RIntCnt_Val : Outport  Port=129  OutDataTypeStr=IntCnt  PortDimensions=1
  acsEntryAll4sBwdReq_Val : Outport  Port=130  OutDataTypeStr=boolean  PortDimensions=1
  acsEntryAll4sBwdSoftInt_Val : Outport  Port=131  OutDataTypeStr=IntEnable  PortDimensions=1
  acsEntryAll4sFwdReq_Val : Outport  Port=132  OutDataTypeStr=boolean  PortDimensions=1
  acsEntryAll4sFwdSoftInt_Val : Outport  Port=133  OutDataTypeStr=IntEnable  PortDimensions=1
  acsEntryAll4sBwdReqSig_Val : Outport  Port=134  OutDataTypeStr=boolean  PortDimensions=1
  acsEntryAll4sFwdReqSig_Val : Outport  Port=135  OutDataTypeStr=boolean  PortDimensions=1
  PasReclinerEntryNotf1ChimeEventStat_Val : Outport  Port=136  OutDataTypeStr=boolean  PortDimensions=1
  PasReclinerEntryReq_Val : Outport  Port=137  OutDataTypeStr=boolean  PortDimensions=1
  PasReclinerEntrySoftInt_Val : Outport  Port=138  OutDataTypeStr=IntEnable  PortDimensions=1
  PasReclinerEntrySrcReqTp_Val : Outport  Port=139  OutDataTypeStr=Enum: SrcReqTp1  PortDimensions=1
  PasReclinerExitNotf1ChimeEventStat_Val : Outport  Port=140  OutDataTypeStr=boolean  PortDimensions=1
  PasReclinerExitReq_Val : Outport  Port=141  OutDataTypeStr=boolean  PortDimensions=1
  PasReclinerExitSoftInt_Val : Outport  Port=142  OutDataTypeStr=IntEnable  PortDimensions=1
  PasReclinerExitSrcReqTp_Val : Outport  Port=143  OutDataTypeStr=Enum: SrcReqTp1  PortDimensions=1
  Unfold3LNotf1ChimeEventStat_Val : Outport  Port=144  OutDataTypeStr=boolean  PortDimensions=1
  Unfold3LReq_Val : Outport  Port=145  OutDataTypeStr=boolean  PortDimensions=1
  Unfold3LsrcReqTp_Val : Outport  Port=146  OutDataTypeStr=Enum: SrcReqTp1  PortDimensions=1
  Unfold3RNotf1ChimeEventStat_Val : Outport  Port=147  OutDataTypeStr=boolean  PortDimensions=1
  Unfold3RReq_Val : Outport  Port=148  OutDataTypeStr=boolean  PortDimensions=1
  Unfold3RsrcReqTp_Val : Outport  Port=149  OutDataTypeStr=Enum: SrcReqTp1  PortDimensions=1
  VIPAllOutNotf1ChimeEventStat_Val : Outport  Port=150  OutDataTypeStr=boolean  PortDimensions=1
  VIPAllOutReq_Val : Outport  Port=151  OutDataTypeStr=boolean  PortDimensions=1
  VIPAllOutSoftInt_Val : Outport  Port=152  OutDataTypeStr=IntEnable  PortDimensions=1
  VIPAllOutsrcReqTp_Val : Outport  Port=153  OutDataTypeStr=Enum: SrcReqTp1  PortDimensions=1
  VIPLtOutNotf1ChimeEventStat_Val : Outport  Port=154  OutDataTypeStr=boolean  PortDimensions=1
  VIPLtOutReq_Val : Outport  Port=155  OutDataTypeStr=boolean  PortDimensions=1
  VIPLtOutSoftInt_Val : Outport  Port=156  OutDataTypeStr=IntEnable  PortDimensions=1
  VIPLtOutsrcReqTp_Val : Outport  Port=157  OutDataTypeStr=Enum: SrcReqTp1  PortDimensions=1
  VIPRtOutNotf1ChimeEventStat_Val : Outport  Port=158  OutDataTypeStr=boolean  PortDimensions=1
  VIPRtOutReq_Val : Outport  Port=159  OutDataTypeStr=boolean  PortDimensions=1
  VIPRtOutSoftInt_Val : Outport  Port=160  OutDataTypeStr=IntEnable  PortDimensions=1
  VIPRtOutsrcReqTp_Val : Outport  Port=161  OutDataTypeStr=Enum: SrcReqTp1  PortDimensions=1
  SwPasReclinerEntryIntCnt_Val : Outport  Port=162  OutDataTypeStr=IntCnt  PortDimensions=1
  SwPasReclinerExitIntCnt_Val : Outport  Port=163  OutDataTypeStr=IntCnt  PortDimensions=1
  SwUnfold3LIntCnt_Val : Outport  Port=164  OutDataTypeStr=IntCnt  PortDimensions=1
  SwUnfold3RIntCnt_Val : Outport  Port=165  OutDataTypeStr=IntCnt  PortDimensions=1
  Big4SeatNotf1ChimeEventStat_Val : Outport  Port=166  OutDataTypeStr=boolean  PortDimensions=1
  Big4SeatReq_Val : Outport  Port=167  OutDataTypeStr=boolean  PortDimensions=1
  Big4SeatSoftInt_Val : Outport  Port=168  OutDataTypeStr=IntEnable  PortDimensions=1
  Big4SeatsrcReqTp_Val : Outport  Port=169  OutDataTypeStr=Enum: SrcReqTp1  PortDimensions=1
  Unfold3LSoftInt_Val : Outport  Port=170  OutDataTypeStr=IntEnable  PortDimensions=1
  Unfold3RSoftInt_Val : Outport  Port=171  OutDataTypeStr=IntEnable  PortDimensions=1
  ExVIPRNotf1ChimeEventStat_Val : Outport  Port=172  OutDataTypeStr=boolean  PortDimensions=1
  ExVIPROutNotf1ChimeEventStat_Val : Outport  Port=173  OutDataTypeStr=boolean  PortDimensions=1
  ExVIPROutReq_Val : Outport  Port=174  OutDataTypeStr=boolean  PortDimensions=1
  ExVIPROutSoftInt_Val : Outport  Port=175  OutDataTypeStr=IntEnable  PortDimensions=1
  ExVIPROutsrcReqTp_Val : Outport  Port=176  OutDataTypeStr=Enum: SrcReqTp1  PortDimensions=1
  ExVIPRReq_Val : Outport  Port=177  OutDataTypeStr=boolean  PortDimensions=1
  ExVIPRSoftInt_Val : Outport  Port=178  OutDataTypeStr=IntEnable  PortDimensions=1
  ExVIPRsrcReqTp_Val : Outport  Port=179  OutDataTypeStr=Enum: SrcReqTp1  PortDimensions=1
  WholeVehMem1Notf1ChimeEventStat_Val : Outport  Port=180  OutDataTypeStr=boolean  PortDimensions=1
  WholeVehMem1Req_Val : Outport  Port=181  OutDataTypeStr=boolean  PortDimensions=1
  WholeVehMem1SoftInt_Val : Outport  Port=182  OutDataTypeStr=IntEnable  PortDimensions=1
  WholeVehMem1srcReqTp_Val : Outport  Port=183  OutDataTypeStr=Enum: SrcReqTp1  PortDimensions=1
  WholeVehMem2Notf1ChimeEventStat_Val : Outport  Port=184  OutDataTypeStr=boolean  PortDimensions=1
  WholeVehMem2Req_Val : Outport  Port=185  OutDataTypeStr=boolean  PortDimensions=1
  WholeVehMem2SoftInt_Val : Outport  Port=186  OutDataTypeStr=IntEnable  PortDimensions=1
  WholeVehMem2srcReqTp_Val : Outport  Port=187  OutDataTypeStr=Enum: SrcReqTp1  PortDimensions=1
  wires:
  AcsEntry2LSwt_Val/1 -> ModelInputHandleRunnable_sys/1(AcsEntry2LSwt_Val_read)
  AcsEntrySwValid_Val/1 -> ModelInputHandleRunnable_sys/2(AcsEntrySwValid_Val_read)
  AcsMdEntyAvl_Val/1 -> ModelInputHandleRunnable_sys/3(AcsMdEntyAvl_Val_read)
  AcsMdEtrySwRtRclReq_Val/1 -> ModelInputHandleRunnable_sys/4(AcsMdEtrySwRtRclReq_Val_read)
  AcsMdEtrySwRtRclReqV_Val/1 -> ModelInputHandleRunnable_sys/5(AcsMdEtrySwRtRclReqV_Val_read)
  AcsMdExtAvl_Val/1 -> ModelInputHandleRunnable_sys/6(AcsMdExtAvl_Val_read)
  AcsMdExtSwLtRclReq_Val/1 -> ModelInputHandleRunnable_sys/7(AcsMdExtSwLtRclReq_Val_read)
  AcsMdExtSwLtRclReqV_Val/1 -> ModelInputHandleRunnable_sys/8(AcsMdExtSwLtRclReqV_Val_read)
  AcsMdExtSwRtRclReq_Val/1 -> ModelInputHandleRunnable_sys/9(AcsMdExtSwRtRclReq_Val_read)
  AcsMdExtSwRtRclReqV_Val/1 -> ModelInputHandleRunnable_sys/10(AcsMdExtSwRtRclReqV_Val_read)
  FamilyMdLtAvl_Val/1 -> ModelInputHandleRunnable_sys/11(FamilyMdLtAvl_Val_read)
  FamilyMdRtAvl_Val/1 -> ModelInputHandleRunnable_sys/12(FamilyMdRtAvl_Val_read)
  HMIMode10RclReq_2R_Val/1 -> ModelInputHandleRunnable_sys/13(HMIMode10RclReq_2R_Val_read)
  HMIMode10RclReq_2L_Val/1 -> ModelInputHandleRunnable_sys/14(HMIMode10RclReq_2L_Val_read)
  HMIMode11RclReq_2R_Val/1 -> ModelInputHandleRunnable_sys/15(HMIMode11RclReq_2R_Val_read)
  HMIMode11RclReq_2L_Val/1 -> ModelInputHandleRunnable_sys/16(HMIMode11RclReq_2L_Val_read)
  HMIMode12RclReq_2R_Val/1 -> ModelInputHandleRunnable_sys/17(HMIMode12RclReq_2R_Val_read)
  HMIMode12RclReq_2L_Val/1 -> ModelInputHandleRunnable_sys/18(HMIMode12RclReq_2L_Val_read)
  HMIMode13RclReq_2R_Val/1 -> ModelInputHandleRunnable_sys/19(HMIMode13RclReq_2R_Val_read)
  HMIMode13RclReq_2L_Val/1 -> ModelInputHandleRunnable_sys/20(HMIMode13RclReq_2L_Val_read)
  HMIMode14RclReq_2R_Val/1 -> ModelInputHandleRunnable_sys/21(HMIMode14RclReq_2R_Val_read)
  HMIMode14RclReq_2L_Val/1 -> ModelInputHandleRunnable_sys/22(HMIMode14RclReq_2L_Val_read)
  HMIMode15RclReq_2R_Val/1 -> ModelInputHandleRunnable_sys/23(HMIMode15RclReq_2R_Val_read)
  HMIMode15RclReq_2L_Val/1 -> ModelInputHandleRunnable_sys/24(HMIMode15RclReq_2L_Val_read)
  HMIMode16RclReq_2R_Val/1 -> ModelInputHandleRunnable_sys/25(HMIMode16RclReq_2R_Val_read)
  HMIMode16RclReq_2L_Val/1 -> ModelInputHandleRunnable_sys/26(HMIMode16RclReq_2L_Val_read)
  HMIMode17RclReq_2R_Val/1 -> ModelInputHandleRunnable_sys/27(HMIMode17RclReq_2R_Val_read)
  HMIMode17RclReq_2L_Val/1 -> ModelInputHandleRunnable_sys/28(HMIMode17RclReq_2L_Val_read)
  HMIMode18RclReq_2R_Val/1 -> ModelInputHandleRunnable_sys/29(HMIMode18RclReq_2R_Val_read)
  HMIMode18RclReq_2L_Val/1 -> ModelInputHandleRunnable_sys/30(HMIMode18RclReq_2L_Val_read)
  HMIMode19RclReq_2R_Val/1 -> ModelInputHandleRunnable_sys/31(HMIMode19RclReq_2R_Val_read)
  HMIMode19RclReq_2L_Val/1 -> ModelInputHandleRunnable_sys/32(HMIMode19RclReq_2L_Val_read)
  HMIMode1RclReq_2R_Val/1 -> ModelInputHandleRunnable_sys/33(HMIMode1RclReq_2R_Val_read)
  HMIMode1RclReq_2L_Val/1 -> ModelInputHandleRunnable_sys/34(HMIMode1RclReq_2L_Val_read)
  HMIMode20RclReq_2R_Val/1 -> ModelInputHandleRunnable_sys/35(HMIMode20RclReq_2R_Val_read)
  HMIMode20RclReq_2L_Val/1 -> ModelInputHandleRunnable_sys/36(HMIMode20RclReq_2L_Val_read)
  HMIMode21RclReq_2R_Val/1 -> ModelInputHandleRunnable_sys/37(HMIMode21RclReq_2R_Val_read)
  HMIMode21RclReq_2L_Val/1 -> ModelInputHandleRunnable_sys/38(HMIMode21RclReq_2L_Val_read)
  HMIMode22RclReq_2R_Val/1 -> ModelInputHandleRunnable_sys/39(HMIMode22RclReq_2R_Val_read)
  HMIMode22RclReq_2L_Val/1 -> ModelInputHandleRunnable_sys/40(HMIMode22RclReq_2L_Val_read)
  HMIMode23RclReq_2R_Val/1 -> ModelInputHandleRunnable_sys/41(HMIMode23RclReq_2R_Val_read)
  HMIMode23RclReq_2L_Val/1 -> ModelInputHandleRunnable_sys/42(HMIMode23RclReq_2L_Val_read)
  HMIMode24RclReq_2R_Val/1 -> ModelInputHandleRunnable_sys/43(HMIMode24RclReq_2R_Val_read)
  HMIMode24RclReq_2L_Val/1 -> ModelInputHandleRunnable_sys/44(HMIMode24RclReq_2L_Val_read)
  HMIMode25RclReq_2R_Val/1 -> ModelInputHandleRunnable_sys/45(HMIMode25RclReq_2R_Val_read)
  HMIMode25RclReq_2L_Val/1 -> ModelInputHandleRunnable_sys/46(HMIMode25RclReq_2L_Val_read)
  HMIMode26RclReq_2R_Val/1 -> ModelInputHandleRunnable_sys/47(HMIMode26RclReq_2R_Val_read)
  HMIMode26RclReq_2L_Val/1 -> ModelInputHandleRunnable_sys/48(HMIMode26RclReq_2L_Val_read)
  HMIMode27RclReq_2R_Val/1 -> ModelInputHandleRunnable_sys/49(HMIMode27RclReq_2R_Val_read)
  HMIMode27RclReq_2L_Val/1 -> ModelInputHandleRunnable_sys/50(HMIMode27RclReq_2L_Val_read)
  HMIMode28RclReq_2R_Val/1 -> ModelInputHandleRunnable_sys/51(HMIMode28RclReq_2R_Val_read)
  HMIMode28RclReq_2L_Val/1 -> ModelInputHandleRunnable_sys/52(HMIMode28RclReq_2L_Val_read)
  HMIMode29RclReq_2R_Val/1 -> ModelInputHandleRunnable_sys/53(HMIMode29RclReq_2R_Val_read)
  HMIMode29RclReq_2L_Val/1 -> ModelInputHandleRunnable_sys/54(HMIMode29RclReq_2L_Val_read)
  HMIMode2RclReq_2R_Val/1 -> ModelInputHandleRunnable_sys/55(HMIMode2RclReq_2R_Val_read)
  HMIMode2RclReq_2L_Val/1 -> ModelInputHandleRunnable_sys/56(HMIMode2RclReq_2L_Val_read)
  HMIMode30RclReq_2R_Val/1 -> ModelInputHandleRunnable_sys/57(HMIMode30RclReq_2R_Val_read)
  HMIMode30RclReq_2L_Val/1 -> ModelInputHandleRunnable_sys/58(HMIMode30RclReq_2L_Val_read)
  HMIMode31RclReq_2R_Val/1 -> ModelInputHandleRunnable_sys/59(HMIMode31RclReq_2R_Val_read)
  HMIMode31RclReq_2L_Val/1 -> ModelInputHandleRunnable_sys/60(HMIMode31RclReq_2L_Val_read)
  HMIMode32RclReq_2R_Val/1 -> ModelInputHandleRunnable_sys/61(HMIMode32RclReq_2R_Val_read)
  HMIMode32RclReq_2L_Val/1 -> ModelInputHandleRunnable_sys/62(HMIMode32RclReq_2L_Val_read)
  HMIMode3RclReq_2R_Val/1 -> ModelInputHandleRunnable_sys/63(HMIMode3RclReq_2R_Val_read)
  HMIMode3RclReq_2L_Val/1 -> ModelInputHandleRunnable_sys/64(HMIMode3RclReq_2L_Val_read)
  HMIMode4RclReq_2R_Val/1 -> ModelInputHandleRunnable_sys/65(HMIMode4RclReq_2R_Val_read)
  HMIMode4RclReq_2L_Val/1 -> ModelInputHandleRunnable_sys/66(HMIMode4RclReq_2L_Val_read)
  HMIMode5RclReq_2R_Val/1 -> ModelInputHandleRunnable_sys/67(HMIMode5RclReq_2R_Val_read)
  HMIMode5RclReq_2L_Val/1 -> ModelInputHandleRunnable_sys/68(HMIMode5RclReq_2L_Val_read)
  HMIMode6RclReq_2R_Val/1 -> ModelInputHandleRunnable_sys/69(HMIMode6RclReq_2R_Val_read)
  HMIMode6RclReq_2L_Val/1 -> ModelInputHandleRunnable_sys/70(HMIMode6RclReq_2L_Val_read)
  HMIMode7RclReq_2R_Val/1 -> ModelInputHandleRunnable_sys/71(HMIMode7RclReq_2R_Val_read)
  HMIMode7RclReq_2L_Val/1 -> ModelInputHandleRunnable_sys/72(HMIMode7RclReq_2L_Val_read)
  HMIMode8RclReq_2R_Val/1 -> ModelInputHandleRunnable_sys/73(HMIMode8RclReq_2R_Val_read)
  HMIMode8RclReq_2L_Val/1 -> ModelInputHandleRunnable_sys/74(HMIMode8RclReq_2L_Val_read)
  HMIMode9RclReq_2R_Val/1 -> ModelInputHandleRunnable_sys/75(HMIMode9RclReq_2R_Val_read)
  HMIMode9RclReq_2L_Val/1 -> ModelInputHandleRunnable_sys/76(HMIMode9RclReq_2L_Val_read)
  IfVeSMSbRrRcvyMdSwRclReq_Val/1 -> ModelInputHandleRunnable_sys/77(IfVeSMSbRrRcvyMdSwRclReq_Val_read)
  IfVeSMSbRrRcvyMdSwRclReqV_Val/1 -> ModelInputHandleRunnable_sys/78(IfVeSMSbRrRcvyMdSwRclReqV_Val_read)
  IfVeSMSeVipMdSwRtRclReqV_Val/1 -> ModelInputHandleRunnable_sys/79(IfVeSMSeVipMdSwRtRclReqV_Val_read)
  IntimacyLMdAvl_Val/1 -> ModelInputHandleRunnable_sys/80(IntimacyLMdAvl_Val_read)
  IntimacyRMdAvl_Val/1 -> ModelInputHandleRunnable_sys/81(IntimacyRMdAvl_Val_read)
  LgrstCloseLtMdAvl_Val/1 -> ModelInputHandleRunnable_sys/82(LgrstCloseLtMdAvl_Val_read)
  LgrstCloseRtMdAvl_Val/1 -> ModelInputHandleRunnable_sys/83(LgrstCloseRtMdAvl_Val_read)
  LgrstOpenLtMdAvl_Val/1 -> ModelInputHandleRunnable_sys/84(LgrstOpenLtMdAvl_Val_read)
  LgrstOpenRtMdAvl_Val/1 -> ModelInputHandleRunnable_sys/85(LgrstOpenRtMdAvl_Val_read)
  LugMdLtAvl_Val/1 -> ModelInputHandleRunnable_sys/86(LugMdLtAvl_Val_read)
  LugMdRtAvl_Val/1 -> ModelInputHandleRunnable_sys/87(LugMdRtAvl_Val_read)
  LugMdSwRclReq_Val/1 -> ModelInputHandleRunnable_sys/88(LugMdSwRclReq_Val_read)
  LugMdSwRclReqV_Val/1 -> ModelInputHandleRunnable_sys/89(LugMdSwRclReqV_Val_read)
  LyingMdLtAvl_Val/1 -> ModelInputHandleRunnable_sys/90(LyingMdLtAvl_Val_read)
  LyingMdRtAvl_Val/1 -> ModelInputHandleRunnable_sys/91(LyingMdRtAvl_Val_read)
  ModeSrcTp_Val/1 -> ModelInputHandleRunnable_sys/92(ModeSrcTp_Val_read)
  oModeState_Val/1 -> ModelInputHandleRunnable_sys/93(oModeState_Val_read)
  RcvyMdLtAvl_Val/1 -> ModelInputHandleRunnable_sys/94(RcvyMdLtAvl_Val_read)
  RcvyMdRtAvl_Val/1 -> ModelInputHandleRunnable_sys/95(RcvyMdRtAvl_Val_read)
  RcvySwRtReq_Val/1 -> ModelInputHandleRunnable_sys/96(RcvySwRtReq_Val_read)
  RcvySwRtReqV_Val/1 -> ModelInputHandleRunnable_sys/97(RcvySwRtReqV_Val_read)
  Recovery2LSwt_Val/1 -> ModelInputHandleRunnable_sys/98(Recovery2LSwt_Val_read)
  SRSCnfmSwReq_67_2_Val/1 -> ModelInputHandleRunnable_sys/99(SRSCnfmSwReq_67_2_Val_read)
  SRSMode_Val/1 -> ModelInputHandleRunnable_sys/100(SRSMode_Val_read)
  SRSSlctSwReq_Val/1 -> ModelInputHandleRunnable_sys/101(SRSSlctSwReq_Val_read)
  StPassCmprtMdHMIReq_Val/1 -> ModelInputHandleRunnable_sys/102(StPassCmprtMdHMIReq_Val_read)
  StPassCmprtMdHMIReqExt_Val/1 -> ModelInputHandleRunnable_sys/103(StPassCmprtMdHMIReqExt_Val_read)
  StSlctSwReq_Val/1 -> ModelInputHandleRunnable_sys/104(StSlctSwReq_Val_read)
  StSlctSwReqV_Val/1 -> ModelInputHandleRunnable_sys/105(StSlctSwReqV_Val_read)
  StSrvReq_Md1_Val/1 -> ModelInputHandleRunnable_sys/106(StSrvReq_Md1_Val_read)
  StSrvReq_Md10_Val/1 -> ModelInputHandleRunnable_sys/107(StSrvReq_Md10_Val_read)
  StSrvReq_Md11_Val/1 -> ModelInputHandleRunnable_sys/108(StSrvReq_Md11_Val_read)
  StSrvReq_Md12_Val/1 -> ModelInputHandleRunnable_sys/109(StSrvReq_Md12_Val_read)
  StSrvReq_Md13_Val/1 -> ModelInputHandleRunnable_sys/110(StSrvReq_Md13_Val_read)
  StSrvReq_Md14_Val/1 -> ModelInputHandleRunnable_sys/111(StSrvReq_Md14_Val_read)
  StSrvReq_Md15_Val/1 -> ModelInputHandleRunnable_sys/112(StSrvReq_Md15_Val_read)
  StSrvReq_Md16_Val/1 -> ModelInputHandleRunnable_sys/113(StSrvReq_Md16_Val_read)
  StSrvReq_Md17_Val/1 -> ModelInputHandleRunnable_sys/114(StSrvReq_Md17_Val_read)
  StSrvReq_Md18_Val/1 -> ModelInputHandleRunnable_sys/115(StSrvReq_Md18_Val_read)
  StSrvReq_Md19_Val/1 -> ModelInputHandleRunnable_sys/116(StSrvReq_Md19_Val_read)
  StSrvReq_Md2_Val/1 -> ModelInputHandleRunnable_sys/117(StSrvReq_Md2_Val_read)
  StSrvReq_Md20_Val/1 -> ModelInputHandleRunnable_sys/118(StSrvReq_Md20_Val_read)
  StSrvReq_Md21_Val/1 -> ModelInputHandleRunnable_sys/119(StSrvReq_Md21_Val_read)
  StSrvReq_Md22_Val/1 -> ModelInputHandleRunnable_sys/120(StSrvReq_Md22_Val_read)
  StSrvReq_Md23_Val/1 -> ModelInputHandleRunnable_sys/121(StSrvReq_Md23_Val_read)
  StSrvReq_Md24_Val/1 -> ModelInputHandleRunnable_sys/122(StSrvReq_Md24_Val_read)
  StSrvReq_Md25_Val/1 -> ModelInputHandleRunnable_sys/123(StSrvReq_Md25_Val_read)
  StSrvReq_Md26_Val/1 -> ModelInputHandleRunnable_sys/124(StSrvReq_Md26_Val_read)
  StSrvReq_Md27_Val/1 -> ModelInputHandleRunnable_sys/125(StSrvReq_Md27_Val_read)
  StSrvReq_Md28_Val/1 -> ModelInputHandleRunnable_sys/126(StSrvReq_Md28_Val_read)
  StSrvReq_Md29_Val/1 -> ModelInputHandleRunnable_sys/127(StSrvReq_Md29_Val_read)
  StSrvReq_Md3_Val/1 -> ModelInputHandleRunnable_sys/128(StSrvReq_Md3_Val_read)
  StSrvReq_Md30_Val/1 -> ModelInputHandleRunnable_sys/129(StSrvReq_Md30_Val_read)
  StSrvReq_Md31_Val/1 -> ModelInputHandleRunnable_sys/130(StSrvReq_Md31_Val_read)
  StSrvReq_Md32_Val/1 -> ModelInputHandleRunnable_sys/131(StSrvReq_Md32_Val_read)
  StSrvReq_Md4_Val/1 -> ModelInputHandleRunnable_sys/132(StSrvReq_Md4_Val_read)
  StSrvReq_Md5_Val/1 -> ModelInputHandleRunnable_sys/133(StSrvReq_Md5_Val_read)
  StSrvReq_Md6_Val/1 -> ModelInputHandleRunnable_sys/134(StSrvReq_Md6_Val_read)
  StSrvReq_Md7_Val/1 -> ModelInputHandleRunnable_sys/135(StSrvReq_Md7_Val_read)
  StSrvReq_Md8_Val/1 -> ModelInputHandleRunnable_sys/136(StSrvReq_Md8_Val_read)
  StSrvReq_Md9_Val/1 -> ModelInputHandleRunnable_sys/137(StSrvReq_Md9_Val_read)
  Vip2LSwt_Val/1 -> ModelInputHandleRunnable_sys/138(Vip2LSwt_Val_read)
  VipMdLtAvl_Val/1 -> ModelInputHandleRunnable_sys/139(VipMdLtAvl_Val_read)
  VipMdRtAvl_Val/1 -> ModelInputHandleRunnable_sys/140(VipMdRtAvl_Val_read)
  VipMdSwRtRclReq_Val/1 -> ModelInputHandleRunnable_sys/141(VipMdSwRtRclReq_Val_read)
  VipRcvySwValid_Val/1 -> ModelInputHandleRunnable_sys/142(VipRcvySwValid_Val_read)
  ModelInputHandleRunnable_sys/1(acsEntyMdReq_Val_write) -> acsEntyMdReq_Val/1
  ModelInputHandleRunnable_sys/2(acsEntyMdSrcTp_Val_write) -> acsEntyMdSrcTp_Val/1
  ModelInputHandleRunnable_sys/3(acsEntySoftInt_Val_write) -> acsEntySoftInt_Val/1
  ModelInputHandleRunnable_sys/4(acsExtMdReq_Val_write) -> acsExtMdReq_Val/1
  ModelInputHandleRunnable_sys/5(acsExtMdSrcTp_Val_write) -> acsExtMdSrcTp_Val/1
  ModelInputHandleRunnable_sys/6(acsExtSoftInt_Val_write) -> acsExtSoftInt_Val/1
  ModelInputHandleRunnable_sys/7(acsMdEntryNotf1ChimeEventStat_Val_write) -> acsMdEntryNotf1ChimeEventStat_Val/1
  ModelInputHandleRunnable_sys/8(acsMdExtNotf1ChimeEventStat_Val_write) -> acsMdExtNotf1ChimeEventStat_Val/1
  ModelInputHandleRunnable_sys/9(AllLugMdReq_Val_write) -> AllLugMdReq_Val/1
  ModelInputHandleRunnable_sys/10(AllLugSoftInt_Val_write) -> AllLugSoftInt_Val/1
  ModelInputHandleRunnable_sys/11(AllLugSrcReqTp_Val_write) -> AllLugSrcReqTp_Val/1
  ModelInputHandleRunnable_sys/12(AllVipMdReq_Val_write) -> AllVipMdReq_Val/1
  ModelInputHandleRunnable_sys/13(AllVipSoftInt_Val_write) -> AllVipSoftInt_Val/1
  ModelInputHandleRunnable_sys/14(AllVipSrcReqTp_Val_write) -> AllVipSrcReqTp_Val/1
  ModelInputHandleRunnable_sys/15(FamilyMdNotf1ChimeEventStat_Val_write) -> FamilyMdNotf1ChimeEventStat_Val/1
  ModelInputHandleRunnable_sys/16(IntimacyMdNotf1ChimeEventStat_Val_write) -> IntimacyMdNotf1ChimeEventStat_Val/1
  ModelInputHandleRunnable_sys/17(IntimacyLtMdReq_Val_write) -> IntimacyLtMdReq_Val/1
  ModelInputHandleRunnable_sys/18(IntimacyLtMdSrcTp_Val_write) -> IntimacyLtMdSrcTp_Val/1
  ModelInputHandleRunnable_sys/19(IntimacyRtMdReq_Val_write) -> IntimacyRtMdReq_Val/1
  ModelInputHandleRunnable_sys/20(IntimacyRtMdSrcTp_Val_write) -> IntimacyRtMdSrcTp_Val/1
  ModelInputHandleRunnable_sys/21(IntimacyRtSoftInt_Val_write) -> IntimacyRtSoftInt_Val/1
  ModelInputHandleRunnable_sys/22(IntimacyLtSoftInt_Val_write) -> IntimacyLtSoftInt_Val/1
  ModelInputHandleRunnable_sys/23(LtFamilyMdReq_Val_write) -> LtFamilyMdReq_Val/1
  ModelInputHandleRunnable_sys/24(LtFamilySoftInt_Val_write) -> LtFamilySoftInt_Val/1
  ModelInputHandleRunnable_sys/25(LtFamilySrcReqTp_Val_write) -> LtFamilySrcReqTp_Val/1
  ModelInputHandleRunnable_sys/26(LtLyingMdReq_Val_write) -> LtLyingMdReq_Val/1
  ModelInputHandleRunnable_sys/27(LtLyingSoftInt_Val_write) -> LtLyingSoftInt_Val/1
  ModelInputHandleRunnable_sys/28(LtLyingSrcReqTp_Val_write) -> LtLyingSrcReqTp_Val/1
  ModelInputHandleRunnable_sys/29(LgrstCloseLtMdReq_Val_write) -> LgrstCloseLtMdReq_Val/1
  ModelInputHandleRunnable_sys/30(LgrstCloseLtSrcReqTp_Val_write) -> LgrstCloseLtSrcReqTp_Val/1
  ModelInputHandleRunnable_sys/31(LgrstCloseLtSoftInt_Val_write) -> LgrstCloseLtSoftInt_Val/1
  ModelInputHandleRunnable_sys/32(LgrstCloseRtMdReq_Val_write) -> LgrstCloseRtMdReq_Val/1
  ModelInputHandleRunnable_sys/33(LgrstCloseRtSrcReqTp_Val_write) -> LgrstCloseRtSrcReqTp_Val/1
  ModelInputHandleRunnable_sys/34(LgrstCloseRtSoftInt_Val_write) -> LgrstCloseRtSoftInt_Val/1
  ModelInputHandleRunnable_sys/35(LgrstLtMdNotf1ChimeEventStat_Val_write) -> LgrstLtMdNotf1ChimeEventStat_Val/1
  ModelInputHandleRunnable_sys/36(LgrstOpenLtMdReq_Val_write) -> LgrstOpenLtMdReq_Val/1
  ModelInputHandleRunnable_sys/37(LgrstOpenLtSrcReqTp_Val_write) -> LgrstOpenLtSrcReqTp_Val/1
  ModelInputHandleRunnable_sys/38(LgrstOpenLtSoftInt_Val_write) -> LgrstOpenLtSoftInt_Val/1
  ModelInputHandleRunnable_sys/39(LgrstOpenRtMdReq_Val_write) -> LgrstOpenRtMdReq_Val/1
  ModelInputHandleRunnable_sys/40(LgrstOpenRtSrcReqTp_Val_write) -> LgrstOpenRtSrcReqTp_Val/1
  ModelInputHandleRunnable_sys/41(LgrstOpenRtSoftInt_Val_write) -> LgrstOpenRtSoftInt_Val/1
  ModelInputHandleRunnable_sys/42(LgrstRtMdNotf1ChimeEventStat_Val_write) -> LgrstRtMdNotf1ChimeEventStat_Val/1
  ModelInputHandleRunnable_sys/43(LtLugMdReq_Val_write) -> LtLugMdReq_Val/1
  ModelInputHandleRunnable_sys/44(LtLugSoftInt_Val_write) -> LtLugSoftInt_Val/1
  ModelInputHandleRunnable_sys/45(LtLugSrcReqTp_Val_write) -> LtLugSrcReqTp_Val/1
  ModelInputHandleRunnable_sys/46(LtRcvyMdReq_Val_write) -> LtRcvyMdReq_Val/1
  ModelInputHandleRunnable_sys/47(LtRcvySoftInt_Val_write) -> LtRcvySoftInt_Val/1
  ModelInputHandleRunnable_sys/48(LtRcvySrcReqTp_Val_write) -> LtRcvySrcReqTp_Val/1
  ModelInputHandleRunnable_sys/49(LtVipMdReq_Val_write) -> LtVipMdReq_Val/1
  ModelInputHandleRunnable_sys/50(LtVipSoftInt_Val_write) -> LtVipSoftInt_Val/1
  ModelInputHandleRunnable_sys/51(LtVipSrcReqTp_Val_write) -> LtVipSrcReqTp_Val/1
  ModelInputHandleRunnable_sys/52(LugMdNotf1ChimeEventStat_Val_write) -> LugMdNotf1ChimeEventStat_Val/1
  ModelInputHandleRunnable_sys/53(LyingMdNotf1ChimeEventStat_Val_write) -> LyingMdNotf1ChimeEventStat_Val/1
  ModelInputHandleRunnable_sys/54(RcvyMdNotf1ChimeEventStat_Val_write) -> RcvyMdNotf1ChimeEventStat_Val/1
  ModelInputHandleRunnable_sys/55(RtFamilyMdReq_Val_write) -> RtFamilyMdReq_Val/1
  ModelInputHandleRunnable_sys/56(RtFamilySoftInt_Val_write) -> RtFamilySoftInt_Val/1
  ModelInputHandleRunnable_sys/57(RtFamilySrcReqTp_Val_write) -> RtFamilySrcReqTp_Val/1
  ModelInputHandleRunnable_sys/58(RtLugMdReq_Val_write) -> RtLugMdReq_Val/1
  ModelInputHandleRunnable_sys/59(RtLugSoftInt_Val_write) -> RtLugSoftInt_Val/1
  ModelInputHandleRunnable_sys/60(RtLugSrcReqTp_Val_write) -> RtLugSrcReqTp_Val/1
  ModelInputHandleRunnable_sys/61(RtLyingMdReq_Val_write) -> RtLyingMdReq_Val/1
  ModelInputHandleRunnable_sys/62(RtLyingSoftInt_Val_write) -> RtLyingSoftInt_Val/1
  ModelInputHandleRunnable_sys/63(RtLyingSrcReqTp_Val_write) -> RtLyingSrcReqTp_Val/1
  ModelInputHandleRunnable_sys/64(RtRcvyMdReq_Val_write) -> RtRcvyMdReq_Val/1
  ModelInputHandleRunnable_sys/65(RtRcvySoftInt_Val_write) -> RtRcvySoftInt_Val/1
  ModelInputHandleRunnable_sys/66(RtRcvySrcReqTp_Val_write) -> RtRcvySrcReqTp_Val/1
  ModelInputHandleRunnable_sys/67(RtVipMdReq_Val_write) -> RtVipMdReq_Val/1
  ModelInputHandleRunnable_sys/68(RtVipSoftInt_Val_write) -> RtVipSoftInt_Val/1
  ModelInputHandleRunnable_sys/69(RtVipSrcReqTp_Val_write) -> RtVipSrcReqTp_Val/1
  ModelInputHandleRunnable_sys/70(SRSAcsEntyIntCnt_Val_write) -> SRSAcsEntyIntCnt_Val/1
  ModelInputHandleRunnable_sys/71(SRSAcsExtIntCnt_Val_write) -> SRSAcsExtIntCnt_Val/1
  ModelInputHandleRunnable_sys/72(SRSAllLugIntCnt_Val_write) -> SRSAllLugIntCnt_Val/1
  ModelInputHandleRunnable_sys/73(SRSAllVipIntCnt_Val_write) -> SRSAllVipIntCnt_Val/1
  ModelInputHandleRunnable_sys/74(SRSIntimacyLtIntCnt_Val_write) -> SRSIntimacyLtIntCnt_Val/1
  ModelInputHandleRunnable_sys/75(SRSIntimacyRtIntCnt_Val_write) -> SRSIntimacyRtIntCnt_Val/1
  ModelInputHandleRunnable_sys/76(SRSLtFamilyIntCnt_Val_write) -> SRSLtFamilyIntCnt_Val/1
  ModelInputHandleRunnable_sys/77(SRSLtLugIntCnt_Val_write) -> SRSLtLugIntCnt_Val/1
  ModelInputHandleRunnable_sys/78(SRSLtLyingIntCnt_Val_write) -> SRSLtLyingIntCnt_Val/1
  ModelInputHandleRunnable_sys/79(SRSLtRcvyIntCnt_Val_write) -> SRSLtRcvyIntCnt_Val/1
  ModelInputHandleRunnable_sys/80(SRSLtVipIntCnt_Val_write) -> SRSLtVipIntCnt_Val/1
  ModelInputHandleRunnable_sys/81(SRSLgrstCloseLtIntCnt_Val_write) -> SRSLgrstCloseLtIntCnt_Val/1
  ModelInputHandleRunnable_sys/82(SRSLgrstCloseRtIntCnt_Val_write) -> SRSLgrstCloseRtIntCnt_Val/1
  ModelInputHandleRunnable_sys/83(SRSLgrstOpenLtIntCnt_Val_write) -> SRSLgrstOpenLtIntCnt_Val/1
  ModelInputHandleRunnable_sys/84(SRSLgrstOpenRtIntCnt_Val_write) -> SRSLgrstOpenRtIntCnt_Val/1
  ModelInputHandleRunnable_sys/85(SRSRtFamilyIntCnt_Val_write) -> SRSRtFamilyIntCnt_Val/1
  ModelInputHandleRunnable_sys/86(SRSRtLugIntCnt_Val_write) -> SRSRtLugIntCnt_Val/1
  ModelInputHandleRunnable_sys/87(SRSRtLyingIntCnt_Val_write) -> SRSRtLyingIntCnt_Val/1
  ModelInputHandleRunnable_sys/88(SRSRtRcvyIntCnt_Val_write) -> SRSRtRcvyIntCnt_Val/1
  ModelInputHandleRunnable_sys/89(SRSRtVipIntCnt_Val_write) -> SRSRtVipIntCnt_Val/1
  ModelInputHandleRunnable_sys/90(SwAcsEntyBIntCnt_Val_write) -> SwAcsEntyBIntCnt_Val/1
  ModelInputHandleRunnable_sys/91(SwAcsEntyLIntCnt_Val_write) -> SwAcsEntyLIntCnt_Val/1
  ModelInputHandleRunnable_sys/92(SwAcsEntyRIntCnt_Val_write) -> SwAcsEntyRIntCnt_Val/1
  ModelInputHandleRunnable_sys/93(SwAcsExtLIntCnt_Val_write) -> SwAcsExtLIntCnt_Val/1
  ModelInputHandleRunnable_sys/94(SwAcsExtRIntCnt_Val_write) -> SwAcsExtRIntCnt_Val/1
  ModelInputHandleRunnable_sys/95(SwAllLugIntCnt_Val_write) -> SwAllLugIntCnt_Val/1
  ModelInputHandleRunnable_sys/96(SwLfVipIntCnt_Val_write) -> SwLfVipIntCnt_Val/1
  ModelInputHandleRunnable_sys/97(SwLtLugIntCnt_Val_write) -> SwLtLugIntCnt_Val/1
  ModelInputHandleRunnable_sys/98(SwLtRcvyIntCnt_Val_write) -> SwLtRcvyIntCnt_Val/1
  ModelInputHandleRunnable_sys/99(SwRtLugIntCnt_Val_write) -> SwRtLugIntCnt_Val/1
  ModelInputHandleRunnable_sys/100(SwRtRcvyIntCnt_Val_write) -> SwRtRcvyIntCnt_Val/1
  ModelInputHandleRunnable_sys/101(SwRtVipIntCnt_Val_write) -> SwRtVipIntCnt_Val/1
  ModelInputHandleRunnable_sys/102(VipMdNotf1ChimeEventStat_Val_write) -> VipMdNotf1ChimeEventStat_Val/1
  ModelInputHandleRunnable/1 -> ModelInputHandleRunnable_sys/Trigger
  ModelInputHandleRunnable_sys/103(MdSWIntSrc_Val_write) -> MdSWIntSrc_Val/1
  AcsEntry4s2LAvl_Val/1 -> ModelInputHandleRunnable_sys/143(AcsEntry4s2LAvl_Val_read)
  AcsEntry4s2RAvl_Val/1 -> ModelInputHandleRunnable_sys/144(AcsEntry4s2RAvl_Val_read)
  AcsEntryAll4sBwdAvl_Val/1 -> ModelInputHandleRunnable_sys/145(AcsEntryAll4sBwdAvl_Val_read)
  AcsEntryAll4sFwdAvl_Val/1 -> ModelInputHandleRunnable_sys/146(AcsEntryAll4sFwdAvl_Val_read)
  AcsExit4s2LAvl_Val/1 -> ModelInputHandleRunnable_sys/147(AcsExit4s2LAvl_Val_read)
  AcsExit4s2RAvl_Val/1 -> ModelInputHandleRunnable_sys/148(AcsExit4s2RAvl_Val_read)
  AcsMdExt4SSwRtRclReq_Val/1 -> ModelInputHandleRunnable_sys/149(AcsMdExt4SSwRtRclReq_Val_read)
  AcsMdExt4SSwRtRclReqV_Val/1 -> ModelInputHandleRunnable_sys/150(AcsMdExt4SSwRtRclReqV_Val_read)
  EZE4SSwReq_Val/1 -> ModelInputHandleRunnable_sys/151(EZE4SSwReq_Val_read)
  ModelInputHandleRunnable_sys/104(SwAcsEntry4s2LIntCnt_Val_write) -> SwAcsEntry4s2LIntCnt_Val/1
  ModelInputHandleRunnable_sys/105(AcsEntry4s2LNotf1ChimeEventStat_Val_write) -> AcsEntry4s2LNotf1ChimeEventStat_Val/1
  ModelInputHandleRunnable_sys/106(acsEntry4s2LReq_Val_write) -> acsEntry4s2LReq_Val/1
  ModelInputHandleRunnable_sys/107(acsEntry4s2LSoftInt_Val_write) -> acsEntry4s2LSoftInt_Val/1
  ModelInputHandleRunnable_sys/108(acsEntry4s2LSrcTp_Val_write) -> acsEntry4s2LSrcTp_Val/1
  ModelInputHandleRunnable_sys/109(SwAcsEntry4s2RIntCnt_Val_write) -> SwAcsEntry4s2RIntCnt_Val/1
  ModelInputHandleRunnable_sys/110(AcsEntry4s2RNotf1ChimeEventStat_Val_write) -> AcsEntry4s2RNotf1ChimeEventStat_Val/1
  ModelInputHandleRunnable_sys/111(acsEntry4s2RReq_Val_write) -> acsEntry4s2RReq_Val/1
  ModelInputHandleRunnable_sys/112(acsEntry4s2RSoftInt_Val_write) -> acsEntry4s2RSoftInt_Val/1
  ModelInputHandleRunnable_sys/113(acsEntry4s2RSrcTp_Val_write) -> acsEntry4s2RSrcTp_Val/1
  ModelInputHandleRunnable_sys/114(AcsEntryAll4sBwdNotf1ChimeEventStat_Val_write) -> AcsEntryAll4sBwdNotf1ChimeEventStat_Val/1
  ModelInputHandleRunnable_sys/115(AcsEntryAll4sFwdNotf1ChimeEventStat_Val_write) -> AcsEntryAll4sFwdNotf1ChimeEventStat_Val/1
  ModelInputHandleRunnable_sys/116(SwAcsExit4s2LIntCnt_Val_write) -> SwAcsExit4s2LIntCnt_Val/1
  ModelInputHandleRunnable_sys/117(AcsExit4s2LNotf1ChimeEventStat_Val_write) -> AcsExit4s2LNotf1ChimeEventStat_Val/1
  ModelInputHandleRunnable_sys/118(acsExit4s2LReq_Val_write) -> acsExit4s2LReq_Val/1
  ModelInputHandleRunnable_sys/119(acsExit4s2LSoftInt_Val_write) -> acsExit4s2LSoftInt_Val/1
  ModelInputHandleRunnable_sys/120(acsExit4s2LSrcTp_Val_write) -> acsExit4s2LSrcTp_Val/1
  ModelInputHandleRunnable_sys/121(SwAcsExit4s2RIntCnt_Val_write) -> SwAcsExit4s2RIntCnt_Val/1
  ModelInputHandleRunnable_sys/122(AcsExit4s2RNotf1ChimeEventStat_Val_write) -> AcsExit4s2RNotf1ChimeEventStat_Val/1
  ModelInputHandleRunnable_sys/123(acsExit4s2RReq_Val_write) -> acsExit4s2RReq_Val/1
  ModelInputHandleRunnable_sys/124(acsExit4s2RSoftInt_Val_write) -> acsExit4s2RSoftInt_Val/1
  ModelInputHandleRunnable_sys/125(acsExit4s2RSrcTp_Val_write) -> acsExit4s2RSrcTp_Val/1
  ModelInputHandleRunnable_sys/126(SRSAcsEntry4s2LIntCnt_Val_write) -> SRSAcsEntry4s2LIntCnt_Val/1
  ModelInputHandleRunnable_sys/127(SRSAcsEntry4s2RIntCnt_Val_write) -> SRSAcsEntry4s2RIntCnt_Val/1
  ModelInputHandleRunnable_sys/128(SRSAcsExit4s2LIntCnt_Val_write) -> SRSAcsExit4s2LIntCnt_Val/1
  ModelInputHandleRunnable_sys/129(SRSAcsExit4s2RIntCnt_Val_write) -> SRSAcsExit4s2RIntCnt_Val/1
  LckUlckActvtFunc_Val/1 -> ModelInputHandleRunnable_sys/152(LckUlckActvtFunc_Val_read)
  NotSecRowLeSeaOccStat_Val/1 -> ModelInputHandleRunnable_sys/153(NotSecRowLeSeaOccStat_Val_read)
  NotSecRowRtSeaOccStat_Val/1 -> ModelInputHandleRunnable_sys/154(NotSecRowRtSeaOccStat_Val_read)
  SysPwrMd_Val/1 -> ModelInputHandleRunnable_sys/155(SysPwrMd_Val_read)
  SysPwrMdV_Val/1 -> ModelInputHandleRunnable_sys/156(SysPwrMdV_Val_read)
  VehMovState_Val/1 -> ModelInputHandleRunnable_sys/157(VehMovState_Val_read)
  LstLckChange_Val/1 -> ModelInputHandleRunnable_sys/158(LstLckChange_Val_read)
  LstLckFunc_Val/1 -> ModelInputHandleRunnable_sys/159(LstLckFunc_Val_read)
  RLDoorAjarSwAct_Val/1 -> ModelInputHandleRunnable_sys/160(RLDoorAjarSwAct_Val_read)
  RRDoorAjarSwAct_Val/1 -> ModelInputHandleRunnable_sys/161(RRDoorAjarSwAct_Val_read)
  ModelInputHandleRunnable_sys/130(acsEntryAll4sBwdReq_Val_write) -> acsEntryAll4sBwdReq_Val/1
  ModelInputHandleRunnable_sys/131(acsEntryAll4sBwdSoftInt_Val_write) -> acsEntryAll4sBwdSoftInt_Val/1
  ModelInputHandleRunnable_sys/132(acsEntryAll4sFwdReq_Val_write) -> acsEntryAll4sFwdReq_Val/1
  ModelInputHandleRunnable_sys/133(acsEntryAll4sFwdSoftInt_Val_write) -> acsEntryAll4sFwdSoftInt_Val/1
  IfVeSMSeStNumConfig_Val/1 -> ModelInputHandleRunnable_sys/162(IfVeSMSeStNumConfig_Val_read)
  PasReclinerAvl_Val/1 -> ModelInputHandleRunnable_sys/163(PasReclinerAvl_Val_read)
  PassStFldDnMovSwAct_Val/1 -> ModelInputHandleRunnable_sys/164(PassStFldDnMovSwAct_Val_read)
  PassStFldDnMovSwActV_Val/1 -> ModelInputHandleRunnable_sys/165(PassStFldDnMovSwActV_Val_read)
  PassStFldUpMovSwAct_Val/1 -> ModelInputHandleRunnable_sys/166(PassStFldUpMovSwAct_Val_read)
  PassStFldUpMovSwActV_Val/1 -> ModelInputHandleRunnable_sys/167(PassStFldUpMovSwActV_Val_read)
  ThdRLtStExpdSwReq_Val/1 -> ModelInputHandleRunnable_sys/168(ThdRLtStExpdSwReq_Val_read)
  ThdRLtStExpdSwReqV_Val/1 -> ModelInputHandleRunnable_sys/169(ThdRLtStExpdSwReqV_Val_read)
  ThdRRtStExpdSwReq_Val/1 -> ModelInputHandleRunnable_sys/170(ThdRRtStExpdSwReq_Val_read)
  ThdRRtStExpdSwReqV_Val/1 -> ModelInputHandleRunnable_sys/171(ThdRRtStExpdSwReqV_Val_read)
  unfold3LAvl_Val/1 -> ModelInputHandleRunnable_sys/172(unfold3LAvl_Val_read)
  unfold3RAvl_Val/1 -> ModelInputHandleRunnable_sys/173(unfold3RAvl_Val_read)
  VipLtOutMdAvl_Val/1 -> ModelInputHandleRunnable_sys/174(VipLtOutMdAvl_Val_read)
  VipRtOutMdAvl_Val/1 -> ModelInputHandleRunnable_sys/175(VipRtOutMdAvl_Val_read)
  ModelInputHandleRunnable_sys/134(acsEntryAll4sBwdReqSig_Val_write) -> acsEntryAll4sBwdReqSig_Val/1
  ModelInputHandleRunnable_sys/135(acsEntryAll4sFwdReqSig_Val_write) -> acsEntryAll4sFwdReqSig_Val/1
  ModelInputHandleRunnable_sys/136(PasReclinerEntryNotf1ChimeEventStat_Val_write) -> PasReclinerEntryNotf1ChimeEventStat_Val/1
  ModelInputHandleRunnable_sys/137(PasReclinerEntryReq_Val_write) -> PasReclinerEntryReq_Val/1
  ModelInputHandleRunnable_sys/138(PasReclinerEntrySoftInt_Val_write) -> PasReclinerEntrySoftInt_Val/1
  ModelInputHandleRunnable_sys/139(PasReclinerEntrySrcReqTp_Val_write) -> PasReclinerEntrySrcReqTp_Val/1
  ModelInputHandleRunnable_sys/140(PasReclinerExitNotf1ChimeEventStat_Val_write) -> PasReclinerExitNotf1ChimeEventStat_Val/1
  ModelInputHandleRunnable_sys/141(PasReclinerExitReq_Val_write) -> PasReclinerExitReq_Val/1
  ModelInputHandleRunnable_sys/142(PasReclinerExitSoftInt_Val_write) -> PasReclinerExitSoftInt_Val/1
  ModelInputHandleRunnable_sys/143(PasReclinerExitSrcReqTp_Val_write) -> PasReclinerExitSrcReqTp_Val/1
  ModelInputHandleRunnable_sys/144(Unfold3LNotf1ChimeEventStat_Val_write) -> Unfold3LNotf1ChimeEventStat_Val/1
  ModelInputHandleRunnable_sys/145(Unfold3LReq_Val_write) -> Unfold3LReq_Val/1
  ModelInputHandleRunnable_sys/146(Unfold3LsrcReqTp_Val_write) -> Unfold3LsrcReqTp_Val/1
  ModelInputHandleRunnable_sys/147(Unfold3RNotf1ChimeEventStat_Val_write) -> Unfold3RNotf1ChimeEventStat_Val/1
  ModelInputHandleRunnable_sys/148(Unfold3RReq_Val_write) -> Unfold3RReq_Val/1
  ModelInputHandleRunnable_sys/149(Unfold3RsrcReqTp_Val_write) -> Unfold3RsrcReqTp_Val/1
  ModelInputHandleRunnable_sys/150(VIPAllOutNotf1ChimeEventStat_Val_write) -> VIPAllOutNotf1ChimeEventStat_Val/1
  ModelInputHandleRunnable_sys/151(VIPAllOutReq_Val_write) -> VIPAllOutReq_Val/1
  ModelInputHandleRunnable_sys/152(VIPAllOutSoftInt_Val_write) -> VIPAllOutSoftInt_Val/1
  ModelInputHandleRunnable_sys/153(VIPAllOutsrcReqTp_Val_write) -> VIPAllOutsrcReqTp_Val/1
  ModelInputHandleRunnable_sys/154(VIPLtOutNotf1ChimeEventStat_Val_write) -> VIPLtOutNotf1ChimeEventStat_Val/1
  ModelInputHandleRunnable_sys/155(VIPLtOutReq_Val_write) -> VIPLtOutReq_Val/1
  ModelInputHandleRunnable_sys/156(VIPLtOutSoftInt_Val_write) -> VIPLtOutSoftInt_Val/1
  ModelInputHandleRunnable_sys/157(VIPLtOutsrcReqTp_Val_write) -> VIPLtOutsrcReqTp_Val/1
  ModelInputHandleRunnable_sys/158(VIPRtOutNotf1ChimeEventStat_Val_write) -> VIPRtOutNotf1ChimeEventStat_Val/1
  ModelInputHandleRunnable_sys/159(VIPRtOutReq_Val_write) -> VIPRtOutReq_Val/1
  ModelInputHandleRunnable_sys/160(VIPRtOutSoftInt_Val_write) -> VIPRtOutSoftInt_Val/1
  ModelInputHandleRunnable_sys/161(VIPRtOutsrcReqTp_Val_write) -> VIPRtOutsrcReqTp_Val/1
  ModelInputHandleRunnable_sys/162(SwPasReclinerEntryIntCnt_Val_write) -> SwPasReclinerEntryIntCnt_Val/1
  ModelInputHandleRunnable_sys/163(SwPasReclinerExitIntCnt_Val_write) -> SwPasReclinerExitIntCnt_Val/1
  ModelInputHandleRunnable_sys/164(SwUnfold3LIntCnt_Val_write) -> SwUnfold3LIntCnt_Val/1
  ModelInputHandleRunnable_sys/165(SwUnfold3RIntCnt_Val_write) -> SwUnfold3RIntCnt_Val/1
  PasReclinerExitAvl_Val/1 -> ModelInputHandleRunnable_sys/176(PasReclinerExitAvl_Val_read)
  StPassCmprtMdHMIReqExt2_Val/1 -> ModelInputHandleRunnable_sys/177(StPassCmprtMdHMIReqExt2_Val_read)
  ModelInputHandleRunnable_sys/166(Big4SeatNotf1ChimeEventStat_Val_write) -> Big4SeatNotf1ChimeEventStat_Val/1
  ModelInputHandleRunnable_sys/167(Big4SeatReq_Val_write) -> Big4SeatReq_Val/1
  ModelInputHandleRunnable_sys/168(Big4SeatSoftInt_Val_write) -> Big4SeatSoftInt_Val/1
  ModelInputHandleRunnable_sys/169(Big4SeatsrcReqTp_Val_write) -> Big4SeatsrcReqTp_Val/1
  ModelInputHandleRunnable_sys/170(Unfold3LSoftInt_Val_write) -> Unfold3LSoftInt_Val/1
  ModelInputHandleRunnable_sys/171(Unfold3RSoftInt_Val_write) -> Unfold3RSoftInt_Val/1
  ModelInputHandleRunnable_sys/172(ExVIPRNotf1ChimeEventStat_Val_write) -> ExVIPRNotf1ChimeEventStat_Val/1
  ModelInputHandleRunnable_sys/173(ExVIPROutNotf1ChimeEventStat_Val_write) -> ExVIPROutNotf1ChimeEventStat_Val/1
  ModelInputHandleRunnable_sys/174(ExVIPROutReq_Val_write) -> ExVIPROutReq_Val/1
  ModelInputHandleRunnable_sys/175(ExVIPROutSoftInt_Val_write) -> ExVIPROutSoftInt_Val/1
  ModelInputHandleRunnable_sys/176(ExVIPROutsrcReqTp_Val_write) -> ExVIPROutsrcReqTp_Val/1
  ModelInputHandleRunnable_sys/177(ExVIPRReq_Val_write) -> ExVIPRReq_Val/1
  ModelInputHandleRunnable_sys/178(ExVIPRSoftInt_Val_write) -> ExVIPRSoftInt_Val/1
  ModelInputHandleRunnable_sys/179(ExVIPRsrcReqTp_Val_write) -> ExVIPRsrcReqTp_Val/1
  Big4SeatAvl_Val/1 -> ModelInputHandleRunnable_sys/178(Big4SeatAvl_Val_read)
  M61WholeVehMemAvl_Val/1 -> ModelInputHandleRunnable_sys/179(M61WholeVehMemAvl_Val_read)
  M62WholeVehMemAvl_Val/1 -> ModelInputHandleRunnable_sys/180(M62WholeVehMemAvl_Val_read)
  ModelInputHandleRunnable_sys/180(WholeVehMem1Notf1ChimeEventStat_Val_write) -> WholeVehMem1Notf1ChimeEventStat_Val/1
  ModelInputHandleRunnable_sys/181(WholeVehMem1Req_Val_write) -> WholeVehMem1Req_Val/1
  ModelInputHandleRunnable_sys/182(WholeVehMem1SoftInt_Val_write) -> WholeVehMem1SoftInt_Val/1
  ModelInputHandleRunnable_sys/183(WholeVehMem1srcReqTp_Val_write) -> WholeVehMem1srcReqTp_Val/1
  ModelInputHandleRunnable_sys/184(WholeVehMem2Notf1ChimeEventStat_Val_write) -> WholeVehMem2Notf1ChimeEventStat_Val/1
  ModelInputHandleRunnable_sys/185(WholeVehMem2Req_Val_write) -> WholeVehMem2Req_Val/1
  ModelInputHandleRunnable_sys/186(WholeVehMem2SoftInt_Val_write) -> WholeVehMem2SoftInt_Val/1
  ModelInputHandleRunnable_sys/187(WholeVehMem2srcReqTp_Val_write) -> WholeVehMem2srcReqTp_Val/1
